simulink model "SWC_FDC_type"  (R2021b)
settings: Solver=FixedStepDiscrete  StartTime=0.0  StopTime=10.0  FixedStep=0.001  RelTol=1e-3
values from neighbouring files (symbols this model uses):
  DID_VCUKey = uint16(0x0202)    [vcu_local_hdr.m]
  DID_XWD = uint16(513)    [vcu_local_hdr.m]
  DIDLen_DKCKey = uint16(8)    [vcu_local_hdr.m]
  DIDLen_DynoMode = uint16(1)    [vcu_local_hdr.m]
  DIDLen_LFLowPresThre = uint16(1)    [vcu_local_hdr.m]
  DIDLen_LFSensorID = uint16(4)    [vcu_local_hdr.m]
  DIDLen_LRLowPresThre = uint16(1)    [vcu_local_hdr.m]
  DIDLen_LRSensorID = uint16(4)    [vcu_local_hdr.m]
  DIDLen_RFLowPresThre = uint16(1)    [vcu_local_hdr.m]
  DIDLen_RFSensorID = uint16(4)    [vcu_local_hdr.m]
  DIDLen_RRLowPresThre = uint16(1)    [vcu_local_hdr.m]
  DIDLen_RRSensorID = uint16(4)    [vcu_local_hdr.m]
  DIDLen_SensorMode = uint16(1)    [vcu_local_hdr.m]
  DIDLen_TPMSLearnSta = uint16(1)    [vcu_local_hdr.m]
  DIDLen_WhlPres = uint16(4)    [vcu_local_hdr.m]
  DIDLen_WhlSensorBattSta = uint16(1)    [vcu_local_hdr.m]
  DIDLen_WhlTmp = uint16(4)    [vcu_local_hdr.m]
  DIDLen_XWDMode = uint16(1)    [vcu_local_hdr.m]
  DIDNum_DKCKey = uint16(0x0202)    [vcu_local_hdr.m]
  DIDNum_DynoMode = uint16(0x0203)    [vcu_local_hdr.m]
  DIDNum_LFLowPresThre = uint16(0x0B08)    [vcu_local_hdr.m]
  DIDNum_LFSensorID = uint16(0x0B01)    [vcu_local_hdr.m]
  DIDNum_LRLowPresThre = uint16(0x0B0A)    [vcu_local_hdr.m]
  DIDNum_LRSensorID = uint16(0x0B03)    [vcu_local_hdr.m]
  DIDNum_RFLowPresThre = uint16(0x0B09)    [vcu_local_hdr.m]
  DIDNum_RFSensorID = uint16(0x0B02)    [vcu_local_hdr.m]
  DIDNum_RRLowPresThre = uint16(0x0B0B)    [vcu_local_hdr.m]
  DIDNum_RRSensorID = uint16(0x0B04)    [vcu_local_hdr.m]
  DIDNum_SensorMode = uint16(0x0B0C)    [vcu_local_hdr.m]
  DIDNum_TPMSLearnSta = uint16(0x0B0D)    [vcu_local_hdr.m]
  DIDNum_WhlPres = uint16(0x0B05)    [vcu_local_hdr.m]
  DIDNum_WhlSensorBattSta = uint16(0x0B07)    [vcu_local_hdr.m]
  DIDNum_WhlTmp = uint16(0x0B06)    [vcu_local_hdr.m]
  DIDNum_XWDMode = uint16(0x0201)    [vcu_local_hdr.m]
  DIDVCUKeyLength = uint16(8)    [vcu_local_hdr.m]
  ENUM_DRIVETRAIN_AWD = uint8(  2  )    [vcu_local_hdr.m]
  ENUM_DRIVETRAIN_FWD = uint8(  1  )    [vcu_local_hdr.m]
  ENUM_DRIVETRAIN_RWD = uint8(  0  )    [vcu_local_hdr.m]
  ENUM_TPMSLearnStatus_LEARNED = uint8(  1  )    [vcu_local_hdr.m]
  ENUM_TPMSLearnStatus_LEARNFAIL = uint8(  2  )    [vcu_local_hdr.m]
  ENUM_TPMSLearnStatus_NOTLEARN = uint8(  0  )    [vcu_local_hdr.m]
  ENUM_TPMSSTA_FAT = uint8(  8  )    [vcu_local_hdr.m]
  ENUM_TPMSSTA_LOWBATTERY = uint8(  2  )    [vcu_local_hdr.m]
  FALSE = boolean( 0 )    [vcu_local_hdr.m]
  ONE_INT = uint8(1)    [vcu_local_hdr.m]
  P_boolean = 0.0    [APPTypes.sldd]
  TRUE = boolean( 1 )    [vcu_local_hdr.m]
  ZERO_FLOAT = single(0)    [vcu_local_hdr.m]
  ZERO_INT = uint8(0)    [vcu_local_hdr.m]
undefined symbols (not defined in the file or in its folder): f32_ApsOutVehSpdSig, KHAL_DKCDecryptEnable_flg_ovrdflg, KHAL_DKCDecryptEnable_flg_ovrdval, KHAL_RandomNumberY1_enum, KHAL_RandomNumberY2_enum, KHAL_RandomNumberY_ovrdflg, KHAL_TPMSRESBUTT_flg_ovrdflg, KHAL_TPMSRESBUTT_flg_ovrdval, R_DIDWriteCDD_CSOP_DIDSet_DKCKey, R_DIDWriteCDD_CSOP_DIDSet_DynoMode, R_DIDWriteCDD_CSOP_DIDSet_LFLowPresThre, R_DIDWriteCDD_CSOP_DIDSet_LFSensorID, R_DIDWriteCDD_CSOP_DIDSet_LRLowPresThre, R_DIDWriteCDD_CSOP_DIDSet_LRSensorID, R_DIDWriteCDD_CSOP_DIDSet_RFLowPresThre, R_DIDWriteCDD_CSOP_DIDSet_RFSensorID, R_DIDWriteCDD_CSOP_DIDSet_RRLowPresThre, R_DIDWriteCDD_CSOP_DIDSet_RRSensorID, R_DIDWriteCDD_CSOP_DIDSet_SensorMode, R_DIDWriteCDD_CSOP_DIDSet_TPMSLearnSta, R_DIDWriteCDD_CSOP_DIDSet_WhlPres, R_DIDWriteCDD_CSOP_DIDSet_WhlSensorBattSta, R_DIDWriteCDD_CSOP_DIDSet_WhlTmp, R_DIDWriteCDD_CSOP_DIDSet_XWDMode, R_E2E_CAN3_VCU1_CSOP_Write_CAN3_VCU1, R_E2E_CAN4_VCU1_CSOP_Write_CAN4_VCU1, R_FDCCDD_Inner_CSOP_FDC_AppCallSleep, R_HALIN_IMU_CSOP_IMUSetSta, R_HALINCDD_CSOP_PAS_Handler, R_HALINCDD_CSOP_UDS_Main, R_HALOUT_APS_CSOP_ApsOutput, R_HALOUTCDD_CSOP_AppNmStateReq, R_HALOUTCDD_CSOP_IVIReset, R_HALOUTCDD_CSOP_SetAcoreRebootCmdACK, R_HALOUTCDD_CSOP_SetSysPwrStat, R_HALOUTCDD_CSOP_SleepRequest, R_NVMReadCDD_Inner_NVM_ReadOperation, R_NVMWriteCDD_Inner_NVM_WriteOperation, R_UDSCDD_CSOP_DdmRestartOperationCycle, R_WDGCDD_CSOP_Call_Watchdog, R_WDGCDD_CSOP_Call_WDG_AppEnd, R_WDGCDD_CSOP_Call_WDG_AppStart, u16_DIDLen_DKCKey, u16_DIDLen_DynoMode, u16_DIDLen_LFLowPresThre, u16_DIDLen_LFSensorID, u16_DIDLen_LRLowPresThre, u16_DIDLen_LRSensorID, u16_DIDLen_RFLowPresThre, u16_DIDLen_RFSensorID, u16_DIDLen_RRLowPresThre, u16_DIDLen_RRSensorID, u16_DIDLen_SensorMode, u16_DIDLen_TPMSLearnSta, u16_DIDLen_WhlPres, u16_DIDLen_WhlSensorBattSta, u16_DIDLen_WhlTmp, u16_DIDLen_XWDMode, u16_DIDNum_DKCKey, u16_DIDNum_DynoMode ... (+42)
libraries: simulink x215, FVT_lib x137, hcu_lib x12, hdlsllib x9, app x1, halin x1, halout x1, inp x1, outp x1
(part 2 of 11)

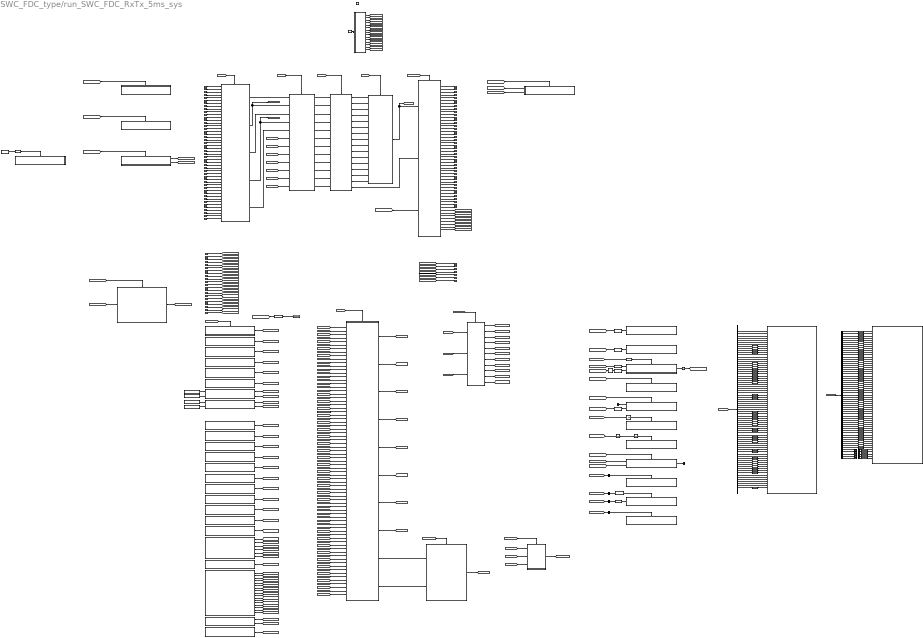
== system SWC_FDC_type/run_SWC_FDC_RxTx_5ms_sys ==
  R_CAN1_ABM1_CAN1_SG_ABM1_read : Inport
  R_CAN1_EPAS1_CAN1_SG_EPAS1_read : Inport  Port=2
  R_CAN1_EPAS2_CAN1_SG_EPAS2_read : Inport  Port=3
  R_CAN1_EPB1_CAN1_SG_EPB1_read : Inport  Port=4
  R_CAN1_ESC1_CAN1_SG_ESC1_read : Inport  Port=5
  R_CAN1_ESC2_CAN1_SG_ESC2_read : Inport  Port=6
  R_CAN1_ESC3_CAN1_SG_ESC3_read : Inport  Port=7
  R_CAN1_ESC4_CAN1_SG_ESC4_read : Inport  Port=8
  R_CAN1_ESC5_CAN1_SG_ESC5_read : Inport  Port=9
  R_CAN1_ESC6_CAN1_SG_ESC6_read : Inport  Port=10
  R_CAN1_ESC7_CAN1_SG_ESC7_read : Inport  Port=11
  R_CAN1_FCM2_CAN1_SG_FCM2_read : Inport  Port=12
  R_CAN1_FCM3_CAN1_SG_FCM3_read : Inport  Port=13
  R_CAN1_FCM4_CAN1_SG_FCM4_read : Inport  Port=14
  R_CAN1_SRR1_CAN1_SG_SRR1_read : Inport  Port=15
  R_CAN2_IVI1_CAN2_SG_IVI1_read : Inport  Port=16
  R_CAN2_IVI2_CAN2_SG_IVI2_read : Inport  Port=17
  R_CAN2_IVI6_CAN2_SG_IVI6_read : Inport  Port=18
  R_CAN2_METER1_CAN2_SG_METER1_read : Inport  Port=19
  R_CAN3_BMS1_CAN3_SG_BMS1_read : Inport  Port=20
  R_CAN3_BMS2_CAN3_SG_BMS2_read : Inport  Port=21
  R_CAN3_BMS3_CAN3_SG_BMS3_read : Inport  Port=22
  R_CAN3_BMS4_CAN3_SG_BMS4_read : Inport  Port=23
  R_CAN3_BMS6_CAN3_SG_BMS6_read : Inport  Port=24
  R_CAN3_BMS7_CAN3_SG_BMS7_read : Inport  Port=25
  R_CAN3_CCU1_CAN3_SG_CCU1_read : Inport  Port=26
  R_CAN3_CCU2_CAN3_SG_CCU2_read : Inport  Port=27
  R_CAN3_CCU4_CAN3_SG_CCU4_read : Inport  Port=28
  R_CAN3_MCU_F1_CAN3_SG_MCU_F1_read : Inport  Port=29
  R_CAN3_MCU_F2_CAN3_SG_MCU_F2_read : Inport  Port=30
  R_CAN3_MCU_R1_CAN3_SG_MCU_R1_read : Inport  Port=31
  R_CAN3_MCU_R2_CAN3_SG_MCU_R2_read : Inport  Port=32
  R_CAN3_Shifter1_CAN3_SG_Shifter1_read : Inport  Port=33
  R_CAN4_DKC1_CAN4_SG_DKC1_read : Inport  Port=34
  R_CAN4_DKC2_CAN4_SG_DKC2_read : Inport  Port=35
  R_CAN4_GW_ZDR_PTG1_CAN4_SG_GW_ZDR_PTG1_read : Inport  Port=36
  R_CAN4_GW_ZoneDR1_CAN4_SG_GW_ZoneDR1_read : Inport  Port=37
  R_CAN4_GW_ZoneDR2_CAN4_SG_GW_ZoneDR2_read : Inport  Port=38
  R_CAN4_GW_ZoneDR3_CAN4_SG_GW_ZoneDR3_read : Inport  Port=39
  R_CAN4_GW_ZoneDR4_CAN4_SG_GW_ZoneDR4_read : Inport  Port=40
  R_CAN4_GW_ZoneDR6_CAN4_SG_GW_ZoneDR6_read : Inport  Port=41
  R_CAN4_GW_ZoneFR1_CAN4_SG_GW_ZoneFR1_read : Inport  Port=42
  R_CAN4_GW_ZoneFR2_CAN4_SG_GW_ZoneFR2_read : Inport  Port=43
  R_CAN4_Zone_Dr_SCP_CAN4_SG_Zone_Dr_SCP_read : Inport  Port=44
  R_CAN4_Zone_Dr_THCM_CAN4_SG_Zone_Dr_THCM_read : Inport  Port=45
  R_CAN4_Zone_Dr_VCU_CAN4_SG_Zone_Dr_VCU_read : Inport  Port=46
  R_CAN4_Zone_Fr_THCM_CAN4_SG_Zone_Fr_THCM_read : Inport  Port=47
  R_CAN5_TBOX1_CAN5_SG_TBOX1_read : Inport  Port=48
  IRV_u16Array4_ApsInDist_read : Inport  Port=49
  IRV_u8Array12_ApsInUssSta_read : Inport  Port=50
  IRV_u8Array256_NvmReadArray_read : Inport  Port=51
  IRV_u8Array8_ApsInLevel_read : Inport  Port=52
  IRV_u8Array8_PasInDist_read : Inport  Port=53
  IRV_u8Array9_TPMSData_read : Inport  Port=54
  IRV_u8_ApsInPASChime_read : Inport  Port=55
  IRV_u8_ApsInSensorLayout_read : Inport  Port=56
  IRV_u8_ApsInSysFailSta_read : Inport  Port=57
  IRV_u8_ApsInSysMode_read : Inport  Port=58
  IRV_u8_CTDSW_read : Inport  Port=59
  IRV_u8_CrashSignal_read : Inport  Port=60
  IRV_u8_DrDoorSW_read : Inport  Port=61
  IRV_u8_HazardSW_read : Inport  Port=62
  IRV_u8_HoodSW_read : Inport  Port=63
  IRV_u8_PsDoorSW_read : Inport  Port=64
  IRV_u8_RLDoorSW_read : Inport  Port=65
  IRV_u8_RRDoorSW_read : Inport  Port=66
  IRV_u8_SeatSW_read : Inport  Port=67
  IRV_u8_TPMSDataInSta_read : Inport  Port=68
  IRV_u8_TailgateSW_read : Inport  Port=69
  IRV_u8_TrunkHanSW_read : Inport  Port=70
  function : TriggerPort  TriggerType=function-call  VariantControl=(inherit)  SampleTimeType=periodic  SampleTime=-1
  APP : app/APP  SystemSampleTime=-1  VariantActivationTime=update diagram  Latency=0  AutoFrameSizeCalculation=off
  Bus Selector : BusSelector  OutputSignals=VOUTP_EnterNewOperCyc_flg
  Bus Selector1 : BusSelector  OutputSignals=VOUTP_AcoreRebootCmdACK_flg
  Bus Selector2 : BusSelector  OutputSignals=VOUTP_IMUEnaCmd_flg
  Bus Selector3 : BusSelector  OutputSignals=VOUTP_PowerSta_enum,VOUTP_BrkPedalPos_pct,VOUTP_ActAPSPosn_pct,VOUTP_LFRawWhlSpeed_kph,VOUTP_RFRawWhlSpeed_kph,VOUTP_LRRawWhlSpeed_kph,VOUTP_RRRawWhlSpeed_kph,VOUTP_LFRawWhlSpeedV_flg,VOUTP_RFRawWhlSpeedV_flg,VOUTP_LRRawWhlSpeedV_flg,VOUTP_RRRawWhlSpeedV_flg,VOUTP_LFWhlRotDir_enum,VOUTP_RFWhlRotDir_enum,VOUTP_LRWhlRotDir_enum,VOUTP_RRWhlRotDir_enum,VOUTP_LFPulseCountV_flg,VOUTP_RFPulseCountV_flg,VOUTP_LRPulseCountV_flg,VOUTP_RRPulseCountV_flg,VOUTP_LFPulseCount_enum,VOUTP_RFPulseCount_enum,VOUTP_LRPulseCount_enum,VOUTP_RRPulseCount_enum,VOUTP_APSActive_flg,VOUTP_APSCtrlAvail_flg,VOUTP_ShifterHandleCmd_enum,VOUTP_DriIntend_enum,VOUTP_EPSAOIControl_enum,VOUTP_SASAngle_Deg,VOUTP_SASSpeed_degps,VOUTP_SASSpeedValid_flg,VOUTP_SASCAL_flg,VOUTP_SASV_flg,VOUTP_GRADE_Deg,VOUTP_YawRate_degps,VOUTP_LatAccel_Gps,VOUTP_LongAccel_Gps,VOUTP_MCPressure_bar,VOUTP_YawRateV_flg,VOUTP_LatAccelV_flg,VOUTP_LongAccelV_flg,VOUTP_MCPressureV_bar,VOUTP_BrkSwSta_flg,VOUTP_BrkSwV_flg,VOUTP_ESCStandstill_flg,VOUTP_ESCAPSSta_enum,VOUTP_EPBExtReleaseAvail_flg,VOUTP_EPBExtApplyAvail_flg,VOUTP_EPBErrSta_enum,VOUTP_EPBSta_enum,VOUTP_AllDoorSW_flg,VOUTP_HoodSW_flg,VOUTP_TailgateSW_flg,VOUTP_AVMparkingcancel_enum,VOUTP_AVMparkingexcute_enum,VOUTP_AVMParkingmode_enum,VOUTP_AVMErrSTA_flg,VOUTP_IVIStatus_flg,VOUTP_CAASSw_enum,VOUTP_IVIScreen_enum,VOUTP_CAASCtrlAvail_flg,VOUTP_ABSActive_flg,VOUTP_TCSActive_flg,VOUTP_DriverSeatBeltCmd_flg,VOUTP_DrDoorSW_flg,VOUTP_PsDoorSW_flg,VOUTP_RLDoorSW_flg,VOUTP_RRDoorSW_flg,VOUTP_RFPressIndi_enum,VOUTP_LFPressIndi_enum,VOUTP_RRPressIndi_enum,VOUTP_LRPressIndi_enum,VOUTP_sigAmbAirT_C,VOUTP_VehActSpd_kph,VOUTP_CAASActive_flg
  Bus Selector4 : BusSelector  OutputSignals=VOUTP_BrkPedalPosTimeOut_flg,VOUTP_LFRawWhlSpeedTimeOut_flg,VOUTP_RFRawWhlSpeedTimeOut_flg,VOUTP_LRRawWhlSpeedTimeOut_flg,VOUTP_RRRawWhlSpeedTimeOut_flg,VOUTP_LFRawWhlSpeedVTimeOut_flg,VOUTP_RFRawWhlSpeedVTimeOut_flg,VOUTP_LRRawWhlSpeedVTimeOut_flg,VOUTP_RRRawWhlSpeedVTimeOut_flg,VOUTP_LFWhlRotDirTimeOut_flg,VOUTP_RFWhlRotDirTimeOut_flg,VOUTP_LRWhlRotDirTimeOut_flg,VOUTP_RRWhlRotDirTimeOut_flg,VOUTP_LFPulseCountVTimeOut_flg,VOUTP_RFPulseCountVTimeOut_flg,VOUTP_LRPulseCountVTimeOut_flg,VOUTP_RRPulseCountVTimeOut_flg,VOUTP_LFPulseCountTimeOut_flg,VOUTP_RFPulseCountTimeOut_flg,VOUTP_LRPulseCountTimeOut_flg,VOUTP_RRPulseCountTimeOut_flg,VOUTP_ShifterHandleCmdTimeOut_flg,VOUTP_DriIntendTimeOut_flg,VOUTP_EPSAOIControlTimeOut_flg,VOUTP_SASAngleTimeOut_flg,VOUTP_SASSpeedTimeOut_flg,VOUTP_SASSpeedValidTimeOut_flg,VOUTP_SASCALTimeOut_flg,VOUTP_SASVTimeOut_flg,VOUTP_GRADETimeOut_flg,VOUTP_YawRateTimeOut_flg,VOUTP_LatAccelTimeOut_flg,VOUTP_LongAccelTimeOut_flg,VOUTP_MCPressureTimeOut_flg,VOUTP_YawRateVTimeOut_flg,VOUTP_LatAccelVTimeOut_flg,VOUTP_LongAccelVTimeOut_flg,VOUTP_MCPressureVTimeOut_flg,VOUTP_BrkSwStaTimeOut_flg,VOUTP_BrkSwVTimeOut_flg,VOUTP_ESCStandstillTimeOut_flg,VOUTP_ESCAPSStaTimeOut_flg,VOUTP_EPBExtReleaseAvailTimeOut_flg,VOUTP_EPBExtApplyAvailTimeOut_flg,VOUTP_EPBErrStaTimeOut_flg,VOUTP_EPBStaTimeOut_flg,VOUTP_AVMparkingcancelTimeOut_flg,VOUTP_AVMparkingexcuteTimeOut_flg,VOUTP_AVMParkingmodeTimeOut_flg,VOUTP_AVMErrSTATimeOut_flg,VOUTP_IVIStatusTimeOut_flg,VOUTP_CAASSwTimeOut_flg,VOUTP_IVIScreenTimeOut_flg,VOUTP_ABSActiveTimeOut_flg,VOUTP_TCSActiveTimeOut_flg,VOUTP_DriverSeatBeltCmdTimeOut_flg,VOUTP_RFPressIndi_enum,VOUTP_LFPressIndi_enum,VOUTP_RRPressIndi_enum,VOUTP_LRPressIndi_enum,VOUTP_sigAmbAirT_C
  Bus Selector5 : BusSelector  OutputSignals=VOUTP_IMUEnaCmd_flg
  Constant : Constant  Value=DIDVCUKeyLength
  Constant1 : Constant  Value=DID_VCUKey
  Constant2 : Constant  Value=uint16(ONE_INT)
  Constant3 : Constant  Value=DID_XWD
  Constant4 : Constant  Value=TRUE
  Constant5 : Constant  Value=FALSE
  Constant6 : Constant  Value=ONE_INT
  DID_CDDSubsystem : Subsystem
  Data Type Conversion{,1..3,5..13,17..19,21..96,98..106,123} (102 alike) : DataTypeConversion  OutDataTypeStr=uint8
  Data Type Conversion{14..16,20} (4 alike) : DataTypeConversion  OutDataTypeStr=int16
  Data Type Conversion4 : DataTypeConversion  OutDataTypeStr=uint32
  Display : Display
  Ground{,1..5} (6 alike) : Ground
  HALOUT_AFTER : Subsystem
  HAL_IN : halin/HAL_IN  SystemSampleTime=-1  VariantActivationTime=update diagram  Latency=0  AutoFrameSizeCalculation=off
  HAL_OUT : halout/HAL_OUT  SystemSampleTime=-1  VariantActivationTime=update diagram  Latency=0  AutoFrameSizeCalculation=off
  Halin_CDD : Subsystem
      settings: RTWSystemCode=Nonreusable function  RTWFcnNameOpts=Use subsystem name  RTWFileNameOpts=Use subsystem name
  INP : inp/INP  SystemSampleTime=-1  VariantActivationTime=update diagram  Latency=0  AutoFrameSizeCalculation=off
  Latch : hcu_lib/Basic_Blocks/Latch
  NOT : Logic  Operator=NOT  Inputs=1  AllPortsSameDT=off  OutDataTypeStr=boolean
  OUTP : outp/OUTP  SystemSampleTime=-1  VariantActivationTime=update diagram  Latency=0  AutoFrameSizeCalculation=off
  OUTP_AFTER : Subsystem
      settings: RTWSystemCode=Nonreusable function  RTWFcnNameOpts=Use subsystem name  RTWFileNameOpts=Use subsystem name
  R_FDCCDD_Inner_CSOP_FDC_AppCallSleep : Subsystem
  R_HALINCDD_CSOP_CAN1BusOff : FunctionCaller  FunctionPrototype=u8_CAN1BusOff = R_HALINCDD_CSOP_CAN1BusOff()  OutputArgumentSpecifications=uint8(1)
  R_HALINCDD_CSOP_CAN2BusOff : FunctionCaller  FunctionPrototype=u8_CAN2BusOff = R_HALINCDD_CSOP_CAN2BusOff()  OutputArgumentSpecifications=uint8(1)
  R_HALINCDD_CSOP_CAN3BusOff : FunctionCaller  FunctionPrototype=u8_CAN3BusOff = R_HALINCDD_CSOP_CAN3BusOff()  OutputArgumentSpecifications=uint8(1)
  R_HALINCDD_CSOP_CAN4BusOff : FunctionCaller  FunctionPrototype=u8_CAN4BusOff = R_HALINCDD_CSOP_CAN4BusOff()  OutputArgumentSpecifications=uint8(1)
  R_HALINCDD_CSOP_CAN5BusOff : FunctionCaller  FunctionPrototype=u8_CAN5BusOff = R_HALINCDD_CSOP_CAN5BusOff()  OutputArgumentSpecifications=uint8(1)
  R_HALINCDD_CSOP_DIDgetDKCdata : FunctionCaller  FunctionPrototype=[u8_DidStaDKC,u8Array8_DidDataDKC] = R_HALINCDD_CSOP_DIDgetDKCdata(u16_lengthDIDDKC,u16_DIDDKC)  InputArgumentSpecifications=uint16(1), uint16(1)  OutputArgumentSpecifications=uint8(1), uint8([1;1;1;1;1;1;1;1])
  R_HALINCDD_CSOP_DIDgetXWDdata : FunctionCaller  FunctionPrototype=[u8_DidStaXWD,u8_DidDataXWD] = R_HALINCDD_CSOP_DIDgetXWDdata(u16_lengthDIDXWD,u16_DIDXWD)  InputArgumentSpecifications=uint16(1), uint16(1)  OutputArgumentSpecifications=uint8(1), uint8(1)
  R_HALINCDD_CSOP_GetAcoreReadyToSleep : FunctionCaller  FunctionPrototype=s8_AcoreReadyToSleep = R_HALINCDD_CSOP_GetAcoreReadyToSleep()  OutputArgumentSpecifications=int8(1)
  R_HALINCDD_CSOP_GetAcoreRebootCmd : FunctionCaller  FunctionPrototype=u8_AcoreRebootCmd = R_HALINCDD_CSOP_GetAcoreRebootCmd()  OutputArgumentSpecifications=uint8(1)
  R_HALINCDD_CSOP_GetAuxBattVoltage : FunctionCaller  FunctionPrototype=u16_AuxBattVol100mV = R_HALINCDD_CSOP_GetAuxBattVoltage()  OutputArgumentSpecifications=uint16(1)
  R_HALINCDD_CSOP_GetBootReason : FunctionCaller  FunctionPrototype=u8_BootReason = R_HALINCDD_CSOP_GetBootReason()  OutputArgumentSpecifications=uint8(1)
  R_HALINCDD_CSOP_GetEvccAplusPwrUpReq : FunctionCaller  FunctionPrototype=u8_EvccAplusPwrUpReq = R_HALINCDD_CSOP_GetEvccAplusPwrUpReq()  OutputArgumentSpecifications=uint8(1)
  R_HALINCDD_CSOP_GetNmState : FunctionCaller  FunctionPrototype=u8_CurrentNMState = R_HALINCDD_CSOP_GetNmState()  OutputArgumentSpecifications=uint8(1)
  R_HALINCDD_CSOP_GetNvmProtectState : FunctionCaller  FunctionPrototype=u8_NvmProtectSta = R_HALINCDD_CSOP_GetNvmProtectState()  OutputArgumentSpecifications=uint8(1)
  R_HALINCDD_CSOP_GetSWID : FunctionCaller  FunctionPrototype=u8Array33_SWID = R_HALINCDD_CSOP_GetSWID()  OutputArgumentSpecifications=uint8([1;1;1;1;1;1;1;1;1;1;1;1;1;1;1;1;1;1;1;1;1;1;1;1;1;1;1;1;1;1;1;1;1])
  R_HALINCDD_CSOP_GetVinpAllowMoveThdOta : FunctionCaller  FunctionPrototype=u8_AllowMovThdOTA = R_HALINCDD_CSOP_GetVinpAllowMoveThdOta()  OutputArgumentSpecifications=uint8(1)
  R_HALINCDD_CSOP_GetVinpPwrReqOta : FunctionCaller  FunctionPrototype=u8_PwrReqOTA = R_HALINCDD_CSOP_GetVinpPwrReqOta()  OutputArgumentSpecifications=uint8(1)
  R_HALINCDD_CSOP_GetWISR : FunctionCaller  FunctionPrototype=u32_WISR = R_HALINCDD_CSOP_GetWISR()  OutputArgumentSpecifications=uint32(1)
  R_HALINCDD_CSOP_HALINCDD_DIRECT : FunctionCaller  FunctionPrototype=[u8_BrakeSW,u8_BrakeLamp,u16_Pedal1Vol,u16_Pedal2Vol,u16_Pedal1Ref5V,u16_Pedal2Ref5V] = R_HALINCDD_CSOP_HALINCDD_DIRECT()  OutputArgumentSpecifications=uint8(1), uint8(1), uint16(1), uint16(1), uint16(1), uint16(1)
  R_HALINCDD_u8Array4_HWID : FunctionCaller  FunctionPrototype=u8Array4_HWID = R_HALINCDD_u8Array4_HWID()  OutputArgumentSpecifications=uint8([1;1;1;1])
  R_HALIN_APS_CSOP_ApsGetData : FunctionCaller  FunctionPrototype=[u8_GetAPS_Progress_PCT,u8_GetAPS_RQ_Display,u8_GetAPS_SW_Ver,u8_GetAPS_HW_Ver,u8_GetAPS_ExitCondition,f32_GetAPS_Angle_Target,u8_GetAPS_Sta_System,u8_GetAPS_V_Rq_EPAS_Ctrl,u8_GetAPS_Rq_EPAS_Ctrl,u8_GetAPS_Req,f32_GetAPS_DecReq,u8_GetAPS_DecReq_A,f32_GetAPS_SpeedCmd,u8_GetAPS_ShftPosnReq,u8_GetAPS_VMC_Req_A,u8_GetCAAS_Sta,u8_GetCAAS_VMC_Req_A] = R_HALIN_APS_CSOP_ApsGetData()  OutputArgumentSpecifications=uint8(1), uint8(1), uint8(1), uint8(1), uint8(1), single(1), uint8(1), uint8(1), uint8(1), uint8(1), single(1), uint8(1), single(1), uint8(1), uint8(1), uint8(1), uint8(1)
  R_HALIN_IMU_CSOP_IMUGetOffsetVal : Subsystem
  R_HALIN_IMU_CSOP_IMUGetSixAxisVal : FunctionCaller  FunctionPrototype=[s16_IMUSixAxisVal,u8_IMUSixAxisValSta] = R_HALIN_IMU_CSOP_IMUGetSixAxisVal()  OutputArgumentSpecifications=int16([1;1;1;1;1;1]), uint8(1)
  R_HALIN_IMU_CSOP_IMUSetSta : Subsystem
  R_HALOUTCDD_CSOP_AppNmStateReq : Subsystem
  R_HALOUTCDD_CSOP_IVIReset : FunctionCaller  FunctionPrototype=R_HALOUTCDD_CSOP_IVIReset(u8_RstValue)  InputArgumentSpecifications=uint8(1)
  R_HALOUTCDD_CSOP_SetAcoreRebootCmdACK : Subsystem
  R_HALOUTCDD_CSOP_SetSysPwrStat : FunctionCaller  FunctionPrototype=R_HALOUTCDD_CSOP_SetSysPwrStat(u8_SysPwrStat)  InputArgumentSpecifications=uint8(1)
  R_HALOUTCDD_CSOP_SleepRequest : Subsystem
  R_HALOUT_APS_CSOP_ApsSetData : FunctionCaller  FunctionPrototype=R_HALOUT_APS_CSOP_ApsSetData(u8_SetPwrSta,f32_SetBrkPedalPos,f32_SetActAPSPosn,f32_SetLF_RawWhlSpeed,f32_SetRF_RawWhlSpeed,f32_SetLR_RawWhlSpeed,f32_SetRR_RawWhlSpeed,u8_SetLF_RawWhlSpeed_V,u8_SetRF_RawWhlSpeed_V,u8_SetLR_RawWhlSpeed_V,u8_SetRR_RawWhlSpeed_V,u8_SetLF_WhlRotDir,u8_SetRF_WhlRotDir,u8_SetLR_WhlRotDir,u8_SetRR_WhlRotDir,u8_SetLF_PulseCount_V,u8_SetRF_PulseCount_V,u8_SetLR_PulseCount_V,u8_SetRR_PulseCount_V,s16_SetLF_PulseCount,s16_SetRF_PulseCount,s16_SetLR_PulseCount,s16_SetRR_PulseCount,u8_SetAPS_Active,u8_SetAPS_CtrlAvail,u8_SetShifter_Handle_Cmd,u8_SetDriIntend,u8_SetEPS_AOI_Control,f32_SetSAS_Angle,f32_SetSAS_Speed,u8_SetSAS_Speed_Valid,u8_SetSAS_CAL,u8_SetSAS_OK,f32_SetGRADE,f32_SetYawRate,f32_SetLatAccel,f32_SetLongAccel,f32_SetMCPressure,u8_SetYawRate_V,u8_SetLatAccel_V,u8_SetLongAccel_V,u8_SetMCPressure_V,u8_SetBrkSw_Sta,u8_SetBrkSw_V,u8_SetESC_Standstill,u8_SetESC_APS_Sta,u8_SetEPBExtReleaseAvail,u8_SetEPBExtApplyAvail,u8_SetEPBErrSta,u8_SetEPBSta,u8_SetAllDoorSW,u8_SetHoodSW,u8_SetTailgate_SW,u8_SetAVM_parking_cancel,u8_SetAVM_parking_excute,u8_SetAVM_Parking_mode,u8_SetAVM_Err_STA,u8_SetIVI_Status,u8_SetCAAS_Sw,u8_SetIVI_Screen,u8_SetCAAS_CtrlAvail,u8_SetABS_Active,u8_SetTCS_Active,u8_SetDriverSeatBeltCmd,u8_SetDrDoorSW,u8_SetPsDoorSW,u8_SetRLDoorSW,u8_SetRRDoorSW,u8_SetRFPressIndi,u8_SetLFPressIndi,u8_SetRRPressIndi,u8_SetLRPressIndi,f32_SetsigAmbAirT,f32_SetVehActSpd,u8_SetCAAS_Active)  InputArgumentSpecifications=uint8(1), single(1), single(1), single(1), single(1), single(1), single(1), uint8(1), uint8(1), uint8(1), uint8(1), uint8(1), uint8(1), uint8(1), uint8(1), uint8(1), uint8(1), uint8(1), uint8(1), int16(1), int16(1), int16(1), int16(1), uint8(1), uint8(1), uint8(1), uint8(1), uint8(1), single(1), single(1), uint8(1), uint8(1), uint8(1), single(1), single(1), single(1), single(1), single(1), uint8(1), uint8(1), uint8(1), uint8(1), uint8(1), uint8(1), uint8(1), uint8(1), uint8(1), uint8(1), uint8(1), uint8(1), uint8(1), uint8(1), uint8(1), uint8(1), uint8(1), uint8(1), uint8(1), uint8(1), uint8(1), uint8(1), uint8(1), uint8(1), uint8(1), uint8(1), uint8(1), uint8(1), uint8(1), uint8(1), uint8(1), uint8(1), uint8(1), uint8(1), single(1), single(1), uint8(1)
  R_HALOUT_APS_CSOP_ApsSetTimeout : FunctionCaller  FunctionPrototype=R_HALOUT_APS_CSOP_ApsSetTimeout(u8_SetBrkPedalPosTO,u8_SetLF_RawWhlSpeedTO,u8_SetRF_RawWhlSpeedTO,u8_SetLR_RawWhlSpeedTO,u8_SetRR_RawWhlSpeedTO,u8_SetLF_RawWhlSpeed_VTO,u8_SetRF_RawWhlSpeed_VTO,u8_SetLR_RawWhlSpeed_VTO,u8_SetRR_RawWhlSpeed_VTO,u8_SetLF_WhlRotDirTO,u8_SetRF_WhlRotDirTO,u8_SetLR_WhlRotDirTO,u8_SetRR_WhlRotDirTO,u8_SetLF_PulseCount_VTO,u8_SetRF_PulseCount_VTO,u8_SetLR_PulseCount_VTO,u8_SetRR_PulseCount_VTO,u8_SetLF_PulseCountTO,u8_SetRF_PulseCountTO,u8_SetLR_PulseCountTO,u8_SetRR_PulseCountTO,u8_SetShifter_Handle_CmdTO,u8_SetDriIntendTO,u8_SetEPS_AOI_ControlTO,u8_SetSAS_AngleTO,u8_SetSAS_SpeedTO,u8_SetSAS_Speed_ValidTO,u8_SetSAS_CALTO,u8_SetSAS_OKTO,u8_SetGRADETO,u8_SetYawRateTO,u8_SetLatAccelTO,u8_SetLongAccelTO,u8_SetMCPressureTO,u8_SetYawRate_VTO,u8_SetLatAccel_VTO,u8_SetLongAccel_VTO,u8_SetMCPressure_VTO,u8_SetBrkSw_StaTO,u8_SetBrkSw_VTO,u8_SetESC_StandstillTO,u8_SetESC_APS_StaTO,u8_SetEPBExtReleaseAvailTO,u8_SetEPBExtApplyAvailTO,u8_SetEPBErrStaTO,u8_SetEPBStaTO,u8_SetAVM_parking_cancelTO,u8_SetAVM_parking_excuteTO,u8_SetAVM_Parking_modeTO,u8_SetAVM_Err_STATO,u8_SetIVI_StatusTO,u8_SetCAAS_SwTO,u8_SetIVI_ScreenTO,u8_SetABS_ActiveTO,u8_SetTCS_ActiveTO,u8_SetDriverSeatBeltCmdTO,u8_SetRFPressIndiTO,u8_SetLFPressIndiTO,u8_SetRRPressIndiTO,u8_SetLRPressIndiTO,u8_SetsigAmbAirTTO)  InputArgumentSpecifications=uint8(1), uint8(1), uint8(1), uint8(1), uint8(1), uint8(1), uint8(1), uint8(1), uint8(1), uint8(1), uint8(1), uint8(1), uint8(1), uint8(1), uint8(1), uint8(1), uint8(1), uint8(1), uint8(1), uint8(1), uint8(1), uint8(1), uint8(1), uint8(1), uint8(1), uint8(1), uint8(1), uint8(1), uint8(1), uint8(1), uint8(1), uint8(1), uint8(1), uint8(1), uint8(1), uint8(1), uint8(1), uint8(1), uint8(1), uint8(1), uint8(1), uint8(1), uint8(1), uint8(1), uint8(1), uint8(1), uint8(1), uint8(1), uint8(1), uint8(1), uint8(1), uint8(1), uint8(1), uint8(1), uint8(1), uint8(1), uint8(1), uint8(1), uint8(1), uint8(1), uint8(1)
  R_NVMReadCDD_Inner_NVM_ReadOperation : Subsystem
  R_NVMWriteCDD_Inner_NVM_WriteOperation : Subsystem
  R_UDSCDD_CSOP_DdmClearDTCNotification : FunctionCaller  FunctionPrototype=u8_ClearDTCcmd = R_UDSCDD_CSOP_DdmClearDTCNotification()  OutputArgumentSpecifications=uint8(1)
  R_UDSCDD_CSOP_DdmRestartOperationCycle : Subsystem
  R_UDSCDD_CSOP_SetDTCStatus : Subsystem
  R_WDGCDD_CSOP_Call_WDG_AppEnd : Subsystem
  R_WDGCDD_CSOP_Call_WDG_AppStart : Subsystem
  R_WDGCDD_CSOP_Call_Watchdog : Subsystem
  Real_DetectChange : hcu_lib/Basic_Blocks/Real_DetectChange
  Subsystem : Subsystem
  Subsystem1 : Subsystem
  Subsystem2 : Subsystem
  Terminator{,1..5} (6 alike) : Terminator
  Unit Delay{,1..3} (4 alike) : UnitDelay  SampleTime=-1  HasFrameUpgradeWarning=on
  detect_Increase : simulink/Logic and Bit Operations/Detect Increase  vinit=0.0  OutDataTypeStr=boolean
  detect_change : simulink/Logic and Bit Operations/Detect Change  vinit=0  OutDataTypeStr=boolean
  hcu_main_sched : Stateflow chart  TreatAsAtomicUnit=on
  P_CAN1_FD_BCM1_CAN1_SG_FD_BCM1_write : Outport
  P_CAN1_FD_VCU1_CAN1_SG_FD_VCU1_write : Outport  Port=2
  P_CAN1_FD_VCU4_CAN1_SG_FD_VCU4_write : Outport  Port=3
  P_CAN2_FD_BCM1_CAN2_SG_FD_BCM1_write : Outport  Port=4
  P_CAN2_FD_BCM2_CAN2_SG_FD_BCM2_write : Outport  Port=5
  P_CAN2_FD_TPMS1_CAN2_SG_FD_TPMS1_write : Outport  Port=6
  P_CAN2_FD_TPMS2_CAN2_SG_FD_TPMS2_write : Outport  Port=7
  P_CAN2_FD_V2L1_CAN2_SG_FD_V2L1_write : Outport  Port=8
  P_CAN2_FD_VCU0_CAN2_SG_FD_VCU0_write : Outport  Port=9
  P_CAN2_FD_VCU1_CAN2_SG_FD_VCU1_write : Outport  Port=10
  P_CAN2_FD_VCU4_CAN2_SG_FD_VCU4_write : Outport  Port=11
  P_CAN2_FD_VMC1_CAN2_SG_FD_VMC1_write : Outport  Port=12
  P_CAN3_FD_BCM1_CAN3_SG_FD_BCM1_write : Outport  Port=13
  P_CAN3_FD_THCM2_CAN3_SG_FD_THCM2_write : Outport  Port=14
  P_CAN3_FD_V2L1_CAN3_SG_FD_V2L1_write : Outport  Port=15
  P_CAN4_FD_DKC1_CAN4_SG_FD_DKC1_write : Outport  Port=16
  P_CAN4_FD_THCM2_CAN4_SG_FD_THCM2_write : Outport  Port=17
  P_CAN5_FD_BCM1_CAN5_SG_FD_BCM1_write : Outport  Port=18
  P_CAN5_FD_CONN1_CAN5_SG_FD_CONN1_write : Outport  Port=19
  P_CAN5_FD_THCM2_CAN5_SG_FD_THCM2_write : Outport  Port=20
  P_CAN5_FD_VCU0_CAN5_SG_FD_VCU0_write : Outport  Port=21
  P_CAN5_FD_VCU1_CAN5_SG_FD_VCU1_write : Outport  Port=22
  P_CAN5_FD_VCU4_CAN5_SG_FD_VCU4_write : Outport  Port=23
  IRV_ms10_CAN1_SG_FD_APS3_write : Outport  Port=24  OutDataTypeStr=Bus: DT_CAN1_SG_FD_APS3  PortDimensions=1  BusOutputAsStruct=on
  IRV_ms10_CAN1_SG_FD_VCU2_write : Outport  Port=25  OutDataTypeStr=Bus: DT_CAN1_SG_FD_VCU2  PortDimensions=1  BusOutputAsStruct=on
  IRV_ms10_CAN1_SG_FD_VCU3_write : Outport  Port=26  OutDataTypeStr=Bus: DT_CAN1_SG_FD_VCU3  PortDimensions=1  BusOutputAsStruct=on
  IRV_ms10_CAN2_SG_FD_APS3_write : Outport  Port=27  OutDataTypeStr=Bus: DT_CAN2_SG_FD_APS3  PortDimensions=1  BusOutputAsStruct=on
  IRV_ms10_CAN2_SG_FD_VCU2_write : Outport  Port=28  OutDataTypeStr=Bus: DT_CAN2_SG_FD_VCU2  PortDimensions=1  BusOutputAsStruct=on
  IRV_ms10_CAN3_SG_FD_VCU0_write : Outport  Port=29  OutDataTypeStr=Bus: DT_CAN3_SG_FD_VCU0  PortDimensions=1  BusOutputAsStruct=on
  IRV_ms10_CAN3_SG_FD_VCU2_write : Outport  Port=30  OutDataTypeStr=Bus: DT_CAN3_SG_FD_VCU2  PortDimensions=1  BusOutputAsStruct=on
  IRV_ms10_CAN5_SG_FD_VCU3_write : Outport  Port=31  OutDataTypeStr=Bus: DT_CAN5_SG_FD_VCU3  PortDimensions=1  BusOutputAsStruct=on
  IRV_ms100_CAN1_SG_FD_THCM1_write : Outport  Port=32  OutDataTypeStr=Bus: DT_CAN1_SG_FD_THCM1  PortDimensions=1  BusOutputAsStruct=on
  IRV_ms100_CAN2_SG_FD_THCM1_write : Outport  Port=33  OutDataTypeStr=Bus: DT_CAN2_SG_FD_THCM1  PortDimensions=1  BusOutputAsStruct=on
  IRV_ms100_CAN3_SG_FD_THCM1_write : Outport  Port=34  OutDataTypeStr=Bus: DT_CAN3_SG_FD_THCM1  PortDimensions=1  BusOutputAsStruct=on
  IRV_ms100_CAN4_SG_FD_THCM1_write : Outport  Port=35  OutDataTypeStr=Bus: DT_CAN4_SG_FD_THCM1  PortDimensions=1  BusOutputAsStruct=on
  IRV_ms20_CAN1_SG_FD_APS1_write : Outport  Port=36  OutDataTypeStr=Bus: DT_CAN1_SG_FD_APS1  PortDimensions=1  BusOutputAsStruct=on
  IRV_ms20_CAN1_SG_FD_APS2_write : Outport  Port=37  OutDataTypeStr=Bus: DT_CAN1_SG_FD_APS2  PortDimensions=1  BusOutputAsStruct=on
  IRV_ms20_CAN2_SG_FD_APS1_write : Outport  Port=38  OutDataTypeStr=Bus: DT_CAN2_SG_FD_APS1  PortDimensions=1  BusOutputAsStruct=on
  IRV_ms20_CAN2_SG_FD_APS2_write : Outport  Port=39  OutDataTypeStr=Bus: DT_CAN2_SG_FD_APS2  PortDimensions=1  BusOutputAsStruct=on
  IRV_ms500_CAN2_SG_FD_VCU5_write : Outport  Port=40  OutDataTypeStr=Bus: DT_CAN2_SG_FD_VCU5  PortDimensions=1  BusOutputAsStruct=on
  IRV_ms500_CAN5_SG_FD_VCU5_write : Outport  Port=41  OutDataTypeStr=Bus: DT_CAN5_SG_FD_VCU5  PortDimensions=1  BusOutputAsStruct=on
  IRV_ms5000_CAN2_SG_FD_VCU6_write : Outport  Port=42  OutDataTypeStr=Bus: DT_CAN2_SG_FD_VCU6  PortDimensions=1  BusOutputAsStruct=on
  IRV_E2E_CAN3_SG_FD_VCU1_write : Outport  Port=43  OutDataTypeStr=Bus: DT_CAN3_SG_FD_VCU1  PortDimensions=1  BusOutputAsStruct=on
  IRV_E2E_CAN4_SG_FD_VCU1_write : Outport  Port=44  OutDataTypeStr=Bus: DT_CAN4_SG_FD_VCU1  PortDimensions=1  BusOutputAsStruct=on
  IRV_f32_ApsOutVehSpdSig_write : Outport  Port=45  OutDataTypeStr=single  PortDimensions=1
  IRV_u8Array256_NvmWriteArray_write : Outport  Port=46  OutDataTypeStr=uint8  PortDimensions=256
  IRV_u8_ApsOutGearPosnSig_write : Outport  Port=47  OutDataTypeStr=uint8  PortDimensions=1
  IRV_u8_ApsOutSendChrgPlugSta_write : Outport  Port=48  OutDataTypeStr=uint8  PortDimensions=1
  IRV_u8_ApsOutSetFrSensorOnCmd_write : Outport  Port=49  OutDataTypeStr=uint8  PortDimensions=1
  IRV_u8_ApsOutSetFrSensorSwTOCmd_write : Outport  Port=50  OutDataTypeStr=uint8  PortDimensions=1
  IRV_u8_ApsOutSetVehSpdTOCmd_write : Outport  Port=51  OutDataTypeStr=uint8  PortDimensions=1
  wires:
  IRV_u16Array4_ApsInDist_read/1 -> [u16Array4_ApsInDist]
  IRV_u8Array12_ApsInUssSta_read/1 -> [u8Array12_ApsInUssSta]
  IRV_u8Array256_NvmReadArray_read/1 -> [u8Array256_NvmReadArray]
  IRV_u8Array8_ApsInLevel_read/1 -> [u8Array8_ApsInLevel]
  IRV_u8Array8_PasInDist_read/1 -> [u8Array8_PasInDist]
  IRV_u8Array9_TPMSData_read/1 -> [u8Array9_TPMSData]
  IRV_u8_ApsInPASChime_read/1 -> [u8_ApsInPASChime]
  IRV_u8_ApsInSensorLayout_read/1 -> [u8_ApsInSensorLayout]
  IRV_u8_ApsInSysFailSta_read/1 -> [u8_ApsInSysFailSta]
  IRV_u8_ApsInSysMode_read/1 -> [u8_ApsInSysMode]
  IRV_u8_CTDSW_read/1 -> [u8_CTDSW]
  IRV_u8_CrashSignal_read/1 -> [u8_CrashSignal]
  IRV_u8_DrDoorSW_read/1 -> [u8_DrDoorSW]
  IRV_u8_HazardSW_read/1 -> [u8_HazardSW]
  IRV_u8_HoodSW_read/1 -> [u8_HoodSW]
  IRV_u8_PsDoorSW_read/1 -> [u8_PsDoorSW]
  IRV_u8_RLDoorSW_read/1 -> [u8_RLDoorSW]
  IRV_u8_RRDoorSW_read/1 -> [u8_RRDoorSW]
  IRV_u8_SeatSW_read/1 -> [u8_SeatSW]
  IRV_u8_TPMSDataInSta_read/1 -> [u8_TPMSDataInSta]
  IRV_u8_TailgateSW_read/1 -> [u8_TailgateSW]
  IRV_u8_TrunkHanSW_read/1 -> [u8_TrunkHanSW]
  [f32_ApsOutVehSpdSig] -> IRV_f32_ApsOutVehSpdSig_write/1
  [u8Array256_NvmWriteArray] -> IRV_u8Array256_NvmWriteArray_write/1
  [u8_ApsOutGearPosnSig] -> IRV_u8_ApsOutGearPosnSig_write/1
  [u8_ApsOutSendChrgPlugSta] -> IRV_u8_ApsOutSendChrgPlugSta_write/1
  [u8_ApsOutSetFrSensorOnCmd] -> IRV_u8_ApsOutSetFrSensorOnCmd_write/1
  [u8_ApsOutSetFrSensorSwTOCmd] -> IRV_u8_ApsOutSetFrSensorSwTOCmd_write/1
  [u8_ApsOutSetVehSpdTOCmd] -> IRV_u8_ApsOutSetVehSpdTOCmd_write/1
  R_HALINCDD_CSOP_CAN1BusOff/1 -> [u8_CAN1BusOff]
  R_HALINCDD_CSOP_CAN2BusOff/1 -> [u8_CAN2BusOff]
  R_HALINCDD_CSOP_CAN3BusOff/1 -> [u8_CAN3BusOff]
  R_HALINCDD_CSOP_CAN4BusOff/1 -> [u8_CAN4BusOff]
  R_HALINCDD_CSOP_CAN5BusOff/1 -> [u8_CAN5BusOff]
  Constant/1 -> R_HALINCDD_CSOP_DIDgetDKCdata/1
  Constant1/1 -> R_HALINCDD_CSOP_DIDgetDKCdata/2
  R_HALINCDD_CSOP_DIDgetDKCdata/1 -> [u8_DidStaDKC]
  R_HALINCDD_CSOP_DIDgetDKCdata/2 -> [u8Array8_DidDataDKC]
  Constant2/1 -> R_HALINCDD_CSOP_DIDgetXWDdata/1
  Constant3/1 -> R_HALINCDD_CSOP_DIDgetXWDdata/2
  R_HALINCDD_CSOP_DIDgetXWDdata/1 -> [u8_DidStaXWD]
  R_HALINCDD_CSOP_DIDgetXWDdata/2 -> [u8_DidDataXWD]
  R_HALINCDD_CSOP_GetAcoreReadyToSleep/1 -> [s8_AcoreReadyToSleep]
  R_HALINCDD_CSOP_GetAcoreRebootCmd/1 -> [u8_AcoreRebootCmd]
  R_HALINCDD_CSOP_GetAuxBattVoltage/1 -> [u16_AuxBattVol100mV]
  R_HALINCDD_CSOP_GetBootReason/1 -> [u8_BootReason]
  R_HALINCDD_CSOP_GetEvccAplusPwrUpReq/1 -> [u8_EvccAplusPwrUpReq]
  R_HALINCDD_CSOP_GetNmState/1 -> [u8_CurrentNMState]
  R_HALINCDD_CSOP_GetNvmProtectState/1 -> [u8_NvmProtectSta]
  R_HALINCDD_CSOP_GetSWID/1 -> [u8Array33_SWID]
  R_HALINCDD_CSOP_GetVinpAllowMoveThdOta/1 -> [u8_AllowMovThdOTA]
  R_HALINCDD_CSOP_GetVinpPwrReqOta/1 -> [u8_PwrReqOTA]
  R_HALINCDD_CSOP_GetWISR/1 -> [u32_WISR]
  R_HALINCDD_CSOP_HALINCDD_DIRECT/1 -> [u8_BrakeSW]
  R_HALINCDD_CSOP_HALINCDD_DIRECT/2 -> [u8_BrakeLamp]
  R_HALINCDD_CSOP_HALINCDD_DIRECT/3 -> [u16_Pedal1Vol]
  R_HALINCDD_CSOP_HALINCDD_DIRECT/4 -> [u16_Pedal2Vol]
  R_HALINCDD_CSOP_HALINCDD_DIRECT/5 -> [u16_Pedal1Ref5V]
  R_HALINCDD_CSOP_HALINCDD_DIRECT/6 -> [u16_Pedal2Ref5V]
  R_HALINCDD_u8Array4_HWID/1 -> [u8Array4_HWID]
  R_HALIN_APS_CSOP_ApsGetData/1 -> [u8_GetAPS_Progress_PCT]
  R_HALIN_APS_CSOP_ApsGetData/2 -> [u8_GetAPS_RQ_Display]
  R_HALIN_APS_CSOP_ApsGetData/3 -> [u8_GetAPS_SW_Ver]
  R_HALIN_APS_CSOP_ApsGetData/4 -> [u8_GetAPS_HW_Ver]
  R_HALIN_APS_CSOP_ApsGetData/5 -> [u8_GetAPS_ExitCondition]
  R_HALIN_APS_CSOP_ApsGetData/6 -> [f32_GetAPS_Angle_Target]
  R_HALIN_APS_CSOP_ApsGetData/7 -> [u8_GetAPS_Sta_System]
  R_HALIN_APS_CSOP_ApsGetData/8 -> [u8_GetAPS_V_Rq_EPAS_Ctrl]
  R_HALIN_APS_CSOP_ApsGetData/9 -> [u8_GetAPS_Rq_EPAS_Ctrl]
  R_HALIN_APS_CSOP_ApsGetData/10 -> [u8_GetAPS_Req]
  R_HALIN_APS_CSOP_ApsGetData/11 -> [f32_GetAPS_DecReq]
  R_HALIN_APS_CSOP_ApsGetData/12 -> [u8_GetAPS_DecReq_A]
  R_HALIN_APS_CSOP_ApsGetData/13 -> [f32_GetAPS_SpeedCmd]
  R_HALIN_APS_CSOP_ApsGetData/14 -> [u8_GetAPS_ShftPosnReq]
  R_HALIN_APS_CSOP_ApsGetData/15 -> [u8_GetAPS_VMC_Req_A]
  R_HALIN_APS_CSOP_ApsGetData/16 -> [u8_GetCAAS_Sta]
  R_HALIN_APS_CSOP_ApsGetData/17 -> [u8_GetCAAS_VMC_Req_A]
  R_HALIN_IMU_CSOP_IMUGetSixAxisVal/1 -> [s16_IMUSixAxisVal]
  R_HALIN_IMU_CSOP_IMUGetSixAxisVal/2 -> [u8_IMUSixAxisValSta]
  R_UDSCDD_CSOP_DdmClearDTCNotification/1 -> [u8_ClearDTCcmd]
  Data Type Conversion/1 -> R_HALOUTCDD_CSOP_IVIReset/1
  [VOUTP_IVIRST_flg] -> Data Type Conversion/1
  Data Type Conversion1/1 -> R_HALOUTCDD_CSOP_SetSysPwrStat/1
  [VOUTP_SysPowerMode_enum] -> Data Type Conversion1/1
  Data Type Conversion2/1 -> R_HALOUTCDD_CSOP_AppNmStateReq/1(WakeReq)
  [VOUTP_NetworkReq_flg] -> Data Type Conversion2/1
  Data Type Conversion3/1 -> R_HALOUTCDD_CSOP_AppNmStateReq/2(SleepReq)
  NOT/1 -> Data Type Conversion3/1
  [VOUTP_NetworkReq_flg] -> NOT/1
  detect_change/1 -> R_HALOUTCDD_CSOP_AppNmStateReq/Enable
  [VOUTP_NetworkReq_flg] -> detect_change/1
  [VOUTP_NvWriteReqRisingEdge_flg] -> R_NVMWriteCDD_Inner_NVM_WriteOperation/Enable
  Data Type Conversion4/1 -> R_HALOUTCDD_CSOP_SleepRequest/2(WakeUpTime)
  [VOUTP_FdcSlpTime_sec] -> Data Type Conversion4/1
  [VOUTP_FdcSlpReqRisingEdge_flg] -> R_HALOUTCDD_CSOP_SleepRequest/Enable
  Unit Delay/1 -> R_WDGCDD_CSOP_Call_WDG_AppEnd/Enable
  [VOUTP_FdcSlpReqRisingEdge_flg] -> Unit Delay/1
  Unit Delay1/1 -> R_FDCCDD_Inner_CSOP_FDC_AppCallSleep/Enable
  Unit Delay2/1 -> Unit Delay1/1
  [VOUTP_FdcSlpReqRisingEdge_flg] -> Unit Delay2/1
  [Header_Array] -> R_UDSCDD_CSOP_SetDTCStatus/1(Header_Array)
  [DTC_Array] -> R_UDSCDD_CSOP_SetDTCStatus/2(DTC_Array)
  [DTC_Trigger] -> R_UDSCDD_CSOP_SetDTCStatus/Enable
  [trig_Read_NVM_00] -> R_NVMReadCDD_Inner_NVM_ReadOperation/Trigger
  [trig_WDG] -> R_WDGCDD_CSOP_Call_Watchdog/Trigger
  detect_Increase/1 -> R_WDGCDD_CSOP_Call_WDG_AppStart/Enable
  Constant4/1 -> detect_Increase/1
  [trig_ReadIMUOffset_00] -> R_HALIN_IMU_CSOP_IMUGetOffsetVal/Trigger
  R_HALIN_IMU_CSOP_IMUGetOffsetVal/1(Out1) -> [s16_IMUOffsetVal]
  R_HALIN_IMU_CSOP_IMUGetOffsetVal/2(Out2) -> [u8_IMUOffsetValSta]
  [E2E_CAN3_VCU1_Trigger] -> HALOUT_AFTER/1(E2E_CAN3_VCU1_Trigger)
  [E2E_CAN4_VCU1_Trigger] -> HALOUT_AFTER/2(E2E_CAN4_VCU1_Trigger)
  [trig_HAL_OUTAFTER_50_1] -> HALOUT_AFTER/Trigger
  [BOUTP_DIDSetData_outputs] -> DID_CDDSubsystem/1(BOUTP_DIDSetData_outputs)
  [trig_GetDID] -> DID_CDDSubsystem/Trigger
  DID_CDDSubsystem/1(BHAL_DIDGetData_raw) -> [BHAL_DIDGetData_raw]
  hcu_main_sched/3(trig_WDG()) -> [trig_WDG]
  INP/8 -> APP/8
  [trig_HAL_IN_10] -> HAL_IN/Trigger
  HAL_IN/1 -> INP/1
  APP/10 -> OUTP/10
  APP/15 -> OUTP/15
  APP/12 -> OUTP/12
  INP/6 -> APP/6
  OUTP/1 -> [BOUTP_outputs], HAL_OUT/1
  INP/7 -> APP/7
  hcu_main_sched/9(trig_HAL_DKC_10_3()) -> [trig_HAL_DKC_10_3]
  [trig_APP_30] -> APP/Trigger
  INP/12 -> APP/12
  INP/5 -> APP/5
  APP/2 -> OUTP/2
  INP/1 -> APP/1
  [BHAL_APM_outputs] -> INP/9
  INP/2 -> APP/2
  hcu_main_sched/6(trig_HAL_IN_10()) -> [trig_HAL_IN_10]
  [BHAL_SYS_outputs] -> INP/8
  APP/4 -> OUTP/4
  APP/3 -> OUTP/3
  [BHAL_DDM_outputs] -> INP/11
  APP/7 -> OUTP/7
  [BHAL_TPMS_outputs] -> INP/7
  INP/4 -> APP/4
  APP/11 -> OUTP/11
  APP/5 -> OUTP/5
  HAL_IN/4 -> [BHAL_CAN4_outputs], INP/4
  APP/6 -> OUTP/6
  [BHAL_DKC_outputs] -> INP/10
  HAL_IN/3 -> INP/3
  APP/13 -> OUTP/13
  APP/16 -> HAL_OUT/2
  INP/9 -> APP/9
  APP/9 -> OUTP/9
  APP/1 -> OUTP/1
  [trig_INP_20] -> INP/Trigger
  [BHAL_IMU_outputs] -> INP/12
  hcu_main_sched/13(trig_OUTP_AFTER_40_1()) -> [trig_OUTP_AFTER_40_1]
  APP/14 -> OUTP/14
  [trig_HAL_OUT_50] -> HAL_OUT/Trigger
  [s8_AcoreReadyToSleep] -> HAL_OUT/3
  HAL_IN/2 -> INP/2, [BHAL_CAN2_outputs]
  APP/8 -> OUTP/8
  hcu_main_sched/12(trig_OUTP_40()) -> [trig_OUTP_40]
  hcu_main_sched/2(trig_ReadIMUOffset_00()) -> [trig_ReadIMUOffset_00]
  [trig_OUTP_40] -> OUTP/Trigger
  INP/3 -> APP/3
  hcu_main_sched/1(trig_Read_NVM_00()) -> [trig_Read_NVM_00]
  hcu_main_sched/15(trig_HAL_OUTAFTER_50_1()) -> [trig_HAL_OUTAFTER_50_1]
  HAL_IN/5 -> INP/5
  hcu_main_sched/4(trig_GetNMID()) -> [trig_GetNMID]
  hcu_main_sched/14(trig_HAL_OUT_50()) -> [trig_HAL_OUT_50]
  hcu_main_sched/8(trig_HAL_DKC_10_2()) -> [trig_HAL_DKC_10_2]
  INP/11 -> APP/11
  hcu_main_sched/11(trig_APP_30()) -> [trig_APP_30]
  hcu_main_sched/5(trig_GetDID()) -> [trig_GetDID]
  INP/10 -> APP/10
  hcu_main_sched/7(trig_HAL_CDD_10_1()) -> [trig_HAL_CDD_10_1]
  [BHAL_GPIO_outputs] -> INP/6
  hcu_main_sched/10(trig_INP_20()) -> [trig_INP_20]
  Constant5/1 -> hcu_main_sched/1(VHAL_FusionSchedReq_flg)
  R_CAN1_ABM1_CAN1_SG_ABM1_read/1 -> HAL_IN/1
  R_CAN1_EPAS1_CAN1_SG_EPAS1_read/1 -> HAL_IN/2
  R_CAN1_EPAS2_CAN1_SG_EPAS2_read/1 -> HAL_IN/3
  R_CAN1_EPB1_CAN1_SG_EPB1_read/1 -> HAL_IN/4
  R_CAN1_ESC1_CAN1_SG_ESC1_read/1 -> HAL_IN/5
  R_CAN1_ESC2_CAN1_SG_ESC2_read/1 -> HAL_IN/6
  R_CAN1_ESC3_CAN1_SG_ESC3_read/1 -> HAL_IN/7
  R_CAN1_ESC4_CAN1_SG_ESC4_read/1 -> HAL_IN/8
  R_CAN1_ESC5_CAN1_SG_ESC5_read/1 -> HAL_IN/9
  R_CAN1_ESC6_CAN1_SG_ESC6_read/1 -> HAL_IN/10
  R_CAN1_ESC7_CAN1_SG_ESC7_read/1 -> HAL_IN/11
  R_CAN1_FCM2_CAN1_SG_FCM2_read/1 -> HAL_IN/12
  R_CAN1_FCM3_CAN1_SG_FCM3_read/1 -> HAL_IN/13
  R_CAN1_FCM4_CAN1_SG_FCM4_read/1 -> HAL_IN/14
  R_CAN1_SRR1_CAN1_SG_SRR1_read/1 -> HAL_IN/15
  R_CAN2_IVI1_CAN2_SG_IVI1_read/1 -> HAL_IN/16
  R_CAN2_IVI2_CAN2_SG_IVI2_read/1 -> HAL_IN/17
  R_CAN2_IVI6_CAN2_SG_IVI6_read/1 -> HAL_IN/18
  R_CAN2_METER1_CAN2_SG_METER1_read/1 -> HAL_IN/19
  R_CAN3_BMS1_CAN3_SG_BMS1_read/1 -> HAL_IN/20
  R_CAN3_BMS2_CAN3_SG_BMS2_read/1 -> HAL_IN/21
  R_CAN3_BMS3_CAN3_SG_BMS3_read/1 -> HAL_IN/22
  R_CAN3_BMS4_CAN3_SG_BMS4_read/1 -> HAL_IN/23
  R_CAN3_BMS6_CAN3_SG_BMS6_read/1 -> HAL_IN/24
  R_CAN3_BMS7_CAN3_SG_BMS7_read/1 -> HAL_IN/25
  R_CAN3_CCU1_CAN3_SG_CCU1_read/1 -> HAL_IN/26
  R_CAN3_CCU2_CAN3_SG_CCU2_read/1 -> HAL_IN/27
  R_CAN3_CCU4_CAN3_SG_CCU4_read/1 -> HAL_IN/28
  R_CAN3_MCU_F1_CAN3_SG_MCU_F1_read/1 -> HAL_IN/29
  R_CAN3_MCU_F2_CAN3_SG_MCU_F2_read/1 -> HAL_IN/30
  R_CAN3_MCU_R1_CAN3_SG_MCU_R1_read/1 -> HAL_IN/31
  R_CAN3_MCU_R2_CAN3_SG_MCU_R2_read/1 -> HAL_IN/32
  R_CAN3_Shifter1_CAN3_SG_Shifter1_read/1 -> HAL_IN/33
  R_CAN4_DKC1_CAN4_SG_DKC1_read/1 -> HAL_IN/34
  R_CAN4_DKC2_CAN4_SG_DKC2_read/1 -> HAL_IN/35
  R_CAN4_GW_ZDR_PTG1_CAN4_SG_GW_ZDR_PTG1_read/1 -> HAL_IN/36
  R_CAN4_GW_ZoneDR1_CAN4_SG_GW_ZoneDR1_read/1 -> HAL_IN/37
  R_CAN4_GW_ZoneDR2_CAN4_SG_GW_ZoneDR2_read/1 -> HAL_IN/38
  R_CAN4_GW_ZoneDR3_CAN4_SG_GW_ZoneDR3_read/1 -> HAL_IN/39
  R_CAN4_GW_ZoneDR4_CAN4_SG_GW_ZoneDR4_read/1 -> HAL_IN/40
  R_CAN4_GW_ZoneDR6_CAN4_SG_GW_ZoneDR6_read/1 -> HAL_IN/41
  R_CAN4_GW_ZoneFR1_CAN4_SG_GW_ZoneFR1_read/1 -> HAL_IN/42
  R_CAN4_GW_ZoneFR2_CAN4_SG_GW_ZoneFR2_read/1 -> HAL_IN/43
  R_CAN4_Zone_Dr_SCP_CAN4_SG_Zone_Dr_SCP_read/1 -> HAL_IN/44
  R_CAN4_Zone_Dr_THCM_CAN4_SG_Zone_Dr_THCM_read/1 -> HAL_IN/45
  R_CAN4_Zone_Dr_VCU_CAN4_SG_Zone_Dr_VCU_read/1 -> HAL_IN/46
  R_CAN4_Zone_Fr_THCM_CAN4_SG_Zone_Fr_THCM_read/1 -> HAL_IN/47
  R_CAN5_TBOX1_CAN5_SG_TBOX1_read/1 -> HAL_IN/48
  HAL_OUT/1 -> P_CAN1_FD_BCM1_CAN1_SG_FD_BCM1_write/1
  HAL_OUT/2 -> P_CAN1_FD_VCU1_CAN1_SG_FD_VCU1_write/1
  HAL_OUT/3 -> P_CAN1_FD_VCU4_CAN1_SG_FD_VCU4_write/1
  HAL_OUT/4 -> P_CAN2_FD_BCM1_CAN2_SG_FD_BCM1_write/1
  HAL_OUT/5 -> P_CAN2_FD_BCM2_CAN2_SG_FD_BCM2_write/1
  HAL_OUT/6 -> P_CAN2_FD_TPMS1_CAN2_SG_FD_TPMS1_write/1
  HAL_OUT/7 -> P_CAN2_FD_TPMS2_CAN2_SG_FD_TPMS2_write/1
  HAL_OUT/8 -> P_CAN2_FD_V2L1_CAN2_SG_FD_V2L1_write/1
  HAL_OUT/9 -> P_CAN2_FD_VCU0_CAN2_SG_FD_VCU0_write/1
  HAL_OUT/10 -> P_CAN2_FD_VCU1_CAN2_SG_FD_VCU1_write/1
  HAL_OUT/11 -> P_CAN2_FD_VCU4_CAN2_SG_FD_VCU4_write/1
  HAL_OUT/12 -> P_CAN2_FD_VMC1_CAN2_SG_FD_VMC1_write/1
  HAL_OUT/13 -> P_CAN3_FD_BCM1_CAN3_SG_FD_BCM1_write/1
  HAL_OUT/14 -> P_CAN3_FD_THCM2_CAN3_SG_FD_THCM2_write/1
  HAL_OUT/15 -> P_CAN3_FD_V2L1_CAN3_SG_FD_V2L1_write/1
  HAL_OUT/16 -> P_CAN4_FD_DKC1_CAN4_SG_FD_DKC1_write/1
  HAL_OUT/17 -> P_CAN4_FD_THCM2_CAN4_SG_FD_THCM2_write/1
  HAL_OUT/18 -> P_CAN5_FD_BCM1_CAN5_SG_FD_BCM1_write/1
  HAL_OUT/19 -> P_CAN5_FD_CONN1_CAN5_SG_FD_CONN1_write/1
  HAL_OUT/20 -> P_CAN5_FD_THCM2_CAN5_SG_FD_THCM2_write/1
  HAL_OUT/21 -> P_CAN5_FD_VCU0_CAN5_SG_FD_VCU0_write/1
  HAL_OUT/22 -> P_CAN5_FD_VCU1_CAN5_SG_FD_VCU1_write/1
  HAL_OUT/23 -> P_CAN5_FD_VCU4_CAN5_SG_FD_VCU4_write/1
  HAL_OUT/24 -> IRV_ms10_CAN1_SG_FD_APS3_write/1
  HAL_OUT/25 -> IRV_ms10_CAN1_SG_FD_VCU2_write/1
  HAL_OUT/26 -> IRV_ms10_CAN1_SG_FD_VCU3_write/1
  HAL_OUT/27 -> IRV_ms10_CAN2_SG_FD_APS3_write/1
  HAL_OUT/28 -> IRV_ms10_CAN2_SG_FD_VCU2_write/1
  HAL_OUT/29 -> IRV_ms10_CAN3_SG_FD_VCU0_write/1
  HAL_OUT/30 -> IRV_ms10_CAN3_SG_FD_VCU2_write/1
  HAL_OUT/31 -> IRV_ms10_CAN5_SG_FD_VCU3_write/1
  HAL_OUT/32 -> IRV_ms100_CAN1_SG_FD_THCM1_write/1
  HAL_OUT/33 -> IRV_ms100_CAN2_SG_FD_THCM1_write/1
  HAL_OUT/34 -> IRV_ms100_CAN3_SG_FD_THCM1_write/1
  HAL_OUT/35 -> IRV_ms100_CAN4_SG_FD_THCM1_write/1
  HAL_OUT/36 -> IRV_ms20_CAN1_SG_FD_APS1_write/1
  HAL_OUT/37 -> IRV_ms20_CAN1_SG_FD_APS2_write/1
  HAL_OUT/38 -> IRV_ms20_CAN2_SG_FD_APS1_write/1
  HAL_OUT/39 -> IRV_ms20_CAN2_SG_FD_APS2_write/1
  HAL_OUT/40 -> IRV_ms500_CAN2_SG_FD_VCU5_write/1
  HAL_OUT/41 -> IRV_ms500_CAN5_SG_FD_VCU5_write/1
  HAL_OUT/42 -> IRV_ms5000_CAN2_SG_FD_VCU6_write/1
  HAL_OUT/43 -> IRV_E2E_CAN3_SG_FD_VCU1_write/1
  HAL_OUT/44 -> IRV_E2E_CAN4_SG_FD_VCU1_write/1
  HAL_OUT/45 -> [VOUTP_NetworkReq_flg]
  HAL_OUT/46 -> [VOUTP_SysPowerMode_enum]
  HAL_OUT/47 -> [VOUTP_NvWriteReqRisingEdge_flg]
  HAL_OUT/48 -> [VOUTP_FdcSlpReqRisingEdge_flg]
  HAL_OUT/49 -> [VOUTP_FdcSlpTime_sec]
  HAL_OUT/50 -> [VOUTP_IVIRST_flg]
  HAL_OUT/51 -> [E2E_CAN3_VCU1_Trigger]
  HAL_OUT/52 -> [E2E_CAN4_VCU1_Trigger]
  Halin_CDD/7(BHAL_IMU_outputs) -> [BHAL_IMU_outputs]
  Halin_CDD/9(AESKey) -> Subsystem/1(In1)
  [u16_Pedal2Vol] -> Halin_CDD/10(VHAL_AccelPedal2Vol_Raw)
  [Enable_decrypt] -> Subsystem2/1(Enable_Decrypt)
  [trig_HAL_DKC_10_2] -> Subsystem/Trigger
  [u8_PwrReqOTA] -> Halin_CDD/29(VHAL_PwrReq_OTA_enum)
  OUTP_AFTER/8(DTC_Trigger) -> [DTC_Trigger]
  Subsystem2/1(BHAL_DKC_outputs) -> [BHAL_DKC_outputs]
  [u8_ClearDTCcmd] -> Halin_CDD/42(VHAL_ClearDTCcmd_flg)
  [u8Array16_ResultData] -> Subsystem2/2(u8Array16_ResultData)
  OUTP_AFTER/2(ApsOut_SendChrgPlugStaSig) -> [u8_ApsOutSendChrgPlugSta]
  [u8_ApsInSysMode] -> Halin_CDD/8(ModOperationIn)
  [u8_BrakeLamp] -> Halin_CDD/20(VHAL_BrakeLampSW_flg)
  [u8_CurrentNMState] -> Halin_CDD/28(VHAL_CurrentNmState_enum)
  [u8_GetCAAS_Sta] -> Halin_CDD/76(u8_GetCAAS_Sta)
  [u8_GetAPS_ExitCondition] -> Halin_CDD/65(u8_GetAPS_ExitCondition)
  [u8_EvccAplusPwrUpReq] -> Halin_CDD/31(VHAL_EvccAplusPwrUpReq_flg)
  OUTP_AFTER/7(HAL_NvmWriteData_raw) -> [u8Array256_NvmWriteArray]
  OUTP_AFTER/1(ApsOut_GearPosnSig) -> [u8_ApsOutGearPosnSig]
  [u8_GetAPS_Progress_PCT] -> Halin_CDD/61(u8_GetAPS_Progress_PCT)
  [u8_CAN1BusOff] -> Halin_CDD/56(VHAL_CAN1BusOff_raw)
  [u8_CTDSW] -> Halin_CDD/18(VHAL_CentralDoorLockSW_flg)
  Halin_CDD/5(BHAL_SYSTPMS_outputs) -> [BHAL_SYSTPMS_outputs]
  [u8_BootReason] -> Halin_CDD/52(VHAL_PmicBootReason_enum)
  [u8_ApsInSensorLayout] -> Halin_CDD/6(SNSRLayoutIn)
  OUTP_AFTER/3(ApsOut_SetFrSensorOnCmd) -> [u8_ApsOutSetFrSensorOnCmd]
  [BHAL_SYSTPMS_outputs] -> OUTP_AFTER/2(BHAL_SYSTPMS_outputs)
  [u8_HoodSW] -> Halin_CDD/12(VHAL_HoodSW_flg)
  OUTP_AFTER/5(ApsOut_SetVehSpdTOCmd) -> [u8_ApsOutSetVehSpdTOCmd]
  [u8_CAN2BusOff] -> Halin_CDD/57(VHAL_CAN2BusOff_raw)
  [BOUTP_outputs] -> OUTP_AFTER/1(BOUTP_outputs)
  [u16_Pedal1Vol] -> Halin_CDD/9(VHAL_AccelPedal1Vol_Raw)
  OUTP_AFTER/9(Header_Array) -> [Header_Array]
  [u8_GetAPS_HW_Ver] -> Halin_CDD/64(u8_GetAPS_HW_Ver)
  Halin_CDD/10(DKCRawData) -> Subsystem/2(In2)
  [trig_OUTP_AFTER_40_1] -> OUTP_AFTER/Trigger
  Halin_CDD/1(BHAL_APM_outputs) -> [BHAL_APM_outputs]
  [u32_WISR] -> Halin_CDD/53(VHAL_WisrBootReason_raw32)
  [BHAL_CAN4_outputs] -> Subsystem2/3(BHAL_CAN4_outputs)
  Halin_CDD/4(BHAL_TPMS_outputs) -> [BHAL_TPMS_outputs]
  [u8_ApsInSysFailSta] -> Halin_CDD/7(StaFSyaIn)
  [u8_DidStaXWD] -> Halin_CDD/33(VHAL_DidXWDSta_flg)
  [u16_AuxBattVol100mV] -> Halin_CDD/48(VHAL_AuxBattVolmV_100mV)
  [u8_PsDoorSW] -> Halin_CDD/15(VHAL_PsDoorSW_flg)
  [BHAL_DIDGetData_raw] -> Halin_CDD/54(BHAL_DIDGetData_raw)
  Halin_CDD/2(BHAL_GPIO_outputs) -> [BHAL_GPIO_outputs]
  [trig_HAL_DKC_10_3] -> Subsystem2/Trigger
  [u8_GetAPS_RQ_Display] -> Halin_CDD/62(u8_GetAPS_RQ_Display)
  Halin_CDD/6(BHAL_DDM_outputs) -> [BHAL_DDM_outputs]
  [u8Array4_HWID] -> Halin_CDD/24(u8_HWID_4byte)
  [u8_GetAPS_V_Rq_EPAS_Ctrl] -> Halin_CDD/68(u8_GetAPS_V_Rq_EPAS_Ctrl)
  [u8_GetAPS_SW_Ver] -> Halin_CDD/63(u8_GetAPS_SW_Ver)
  [u8_DidStaDKC] -> Halin_CDD/36(VHAL_DIDVCUKeyReadSta_flg)
  [s8_AcoreReadyToSleep] -> Halin_CDD/32(VHAL_AcoreReadyToSlp_flg)
  [u8_GetCAAS_VMC_Req_A] -> Halin_CDD/77(u8_GetCAAS_VMC_Req_A)
  [u8_GetAPS_Sta_System] -> Halin_CDD/67(u8_GetAPS_Sta_System)
  [u8_NvmProtectSta] -> Halin_CDD/47(VHAL_NvmProtectSta_flg)
  [u8Array33_SWID] -> Halin_CDD/26(GetSWID_data)
  [u8Array8_ApsInLevel] -> Halin_CDD/3(APSLevelData)
  [u16_Pedal1Ref5V] -> Halin_CDD/49(VHAL_Pedal1Ref5V_raw)
  [u8_TrunkHanSW] -> Halin_CDD/21(VHAL_TrunkHanSW_flg)
  [u8_RLDoorSW] -> Halin_CDD/17(VHAL_RLDoorSW_flg)
  [u8_AnyNMID] -> Halin_CDD/27(VHAL_AnyNMID_flg)
  [u8_CAN4BusOff] -> Halin_CDD/59(VHAL_CAN4BusOff_raw)
  OUTP_AFTER/10(DTC_Array) -> [DTC_Array]
  [u8_GetAPS_Rq_EPAS_Ctrl] -> Halin_CDD/69(u8_GetAPS_Rq_EPAS_Ctrl)
  [BHAL_SYS_outputs] -> OUTP_AFTER/3(BHAL_SYS_outputs)
  [u8_GetAPS_ShftPosnReq] -> Halin_CDD/74(u8_GetAPS_ShftPosnReq)
  Constant6/1 -> Halin_CDD/25(GetSWID_status)
  [u8_GetAPS_Req] -> Halin_CDD/70(u8_GetAPS_Req)
  [BHAL_CAN2_outputs] -> Halin_CDD/40(BHAL_CAN2_outputs)
  [u8_CrashSignal] -> Halin_CDD/23(VHAL_CrashSignalGPIO_flg)
  [u8_TPMSDataInSta] -> Halin_CDD/38(TPMS_DataIn_flg)
  [u8_IMUOffsetValSta] -> Halin_CDD/45(VHAL_IMUOffsetValSta_flg)
  [u8_HazardSW] -> Halin_CDD/19(VHAL_HazardSW_flg)
  [u8Array256_NvmReadArray] -> Halin_CDD/35(HAL_NvmReadData_raw)
  [u8_AcoreRebootCmd] -> Halin_CDD/55(VHAL_AcoreRebootCmd_raw)
  [u8Array8_PasInDist] -> Halin_CDD/1(PASDistanceData)
  [u8Array12_ApsInUssSta] -> Halin_CDD/4(APSFaultStaData)
  OUTP_AFTER/4(ApsOut_SetFrSensorSwTOCmd) -> [u8_ApsOutSetFrSensorSwTOCmd]
  [s16_IMUSixAxisVal] -> Halin_CDD/44(VHAL_IMUSixAxisVal_raw)
  [u16Array4_ApsInDist] -> Halin_CDD/2(APSDistanceData)
  [u8_RRDoorSW] -> Halin_CDD/16(VHAL_RRDoorSW_flg)
  [f32_GetAPS_SpeedCmd] -> Halin_CDD/73(f32_GetAPS_SpeedCmd)
  [u8_DrDoorSW] -> Halin_CDD/14(VHAL_DrDoorSW_flg)
  [u8_DidDataXWD] -> Halin_CDD/34(VHAL_DidXWDData_enum)
  OUTP_AFTER/6(ApsOut_VehSpdSig) -> [f32_ApsOutVehSpdSig]
  [u8_CAN3BusOff] -> Halin_CDD/58(VHAL_CAN3BusOff_raw)
  [trig_HAL_CDD_10_1] -> Halin_CDD/Trigger
  [u8_BrakeSW] -> Halin_CDD/11(VHAL_BrakeSWGPIO_flg)
  [VHAL_NetworkReqCalled_flg] -> Halin_CDD/51(VHAL_NetworkReqCalled_flg)
  [u8_GetAPS_VMC_Req_A] -> Halin_CDD/75(u8_GetAPS_VMC_Req_A)
  [u8_CAN5BusOff] -> Halin_CDD/60(VHAL_CAN5BusOff_raw)
  [f32_GetAPS_Angle_Target] -> Halin_CDD/66(f32_GetAPS_Angle_Target)
  [u8_ApsInPASChime] -> Halin_CDD/5(ChimeIn)
  [u8_IMUSixAxisValSta] -> Halin_CDD/46(VHAL_IMUSixAxisValSta_flg)
  [u16_Pedal2Ref5V] -> Halin_CDD/50(VHAL_Pedal2Ref5V_raw)
  [u8_SeatSW] -> Halin_CDD/22(VHAL_SeatSW_flg)
  [u8_GetAPS_DecReq_A] -> Halin_CDD/72(u8_GetAPS_DecReq_A)
  OUTP_AFTER/11(BOUTP_DIDSetData_outputs) -> [BOUTP_DIDSetData_outputs]
  [u8Array9_TPMSData] -> Halin_CDD/39(TPMS_RawData)
  [u8_TailgateSW] -> Halin_CDD/13(VHAL_TailgateSW_flg)
  [s16_IMUOffsetVal] -> Halin_CDD/43(VHAL_IMUOffsetVal_raw)
  Subsystem/1(Out1) -> [u8Array16_ResultData]
  [f32_GetAPS_DecReq] -> Halin_CDD/71(f32_GetAPS_DecReq)
  Latch/1 -> Display/1  "VHAL_AnyNMIDLatch_flg"
  [BHAL_CAN4_outputs] -> Halin_CDD/41(BHAL_CAN4_outputs)
  [u8_AllowMovThdOTA] -> Halin_CDD/30(VHAL_AllowMovThd_OTA_enum)
  Halin_CDD/8(Enable_decrypt) -> [Enable_decrypt]
  Halin_CDD/3(BHAL_SYS_outputs) -> [BHAL_SYS_outputs]
  [u8_AnyNMID] -> Latch/1
  [u8Array8_DidDataDKC] -> Halin_CDD/37(VHAL_GetDIDVCUKey_enum)
  Unit Delay3/1 -> [VHAL_NetworkReqCalled_flg]
  R_HALOUTCDD_CSOP_AppNmStateReq/1(Outport) -> Unit Delay3/1
  Real_DetectChange/1 -> R_HALIN_IMU_CSOP_IMUSetSta/Enable
  [BOUTP_outputs] -> Bus Selector1/1
  Bus Selector2/1 -> Data Type Conversion5/1  "<VOUTP_IMUEnaCmd_flg>"
  Bus Selector5/1 -> Real_DetectChange/1  "<VOUTP_IMUEnaCmd_flg>"
  Bus Selector1/1 -> R_HALOUTCDD_CSOP_SetAcoreRebootCmdACK/Enable  "<VOUTP_AcoreRebootCmdACK_flg>"
  [BOUTP_outputs] -> Bus Selector/1
  Data Type Conversion5/1 -> R_HALIN_IMU_CSOP_IMUSetSta/1(u8_IMUEnaCmd)
  Bus Selector/1 -> R_UDSCDD_CSOP_DdmRestartOperationCycle/Enable  "<VOUTP_EnterNewOperCyc_flg>"
  [BOUTP_outputs] -> Bus Selector5/1
  [BOUTP_outputs] -> Bus Selector2/1
  Bus Selector4/32 -> Data Type Conversion65/1  "<VOUTP_LatAccelTimeOut_flg>"
  Data Type Conversion46/1 -> R_HALOUT_APS_CSOP_ApsSetTimeout/14
  Bus Selector4/60 -> Terminator4/1  "<VOUTP_LRPressIndi_enum>"
  Data Type Conversion29/1 -> R_HALOUT_APS_CSOP_ApsSetData/44
  Data Type Conversion103/1 -> R_HALOUT_APS_CSOP_ApsSetData/63
  Bus Selector3/52 -> Data Type Conversion34/1  "<VOUTP_HoodSW_flg>"
  Data Type Conversion72/1 -> R_HALOUT_APS_CSOP_ApsSetTimeout/40
  Data Type Conversion82/1 -> R_HALOUT_APS_CSOP_ApsSetTimeout/47
  Data Type Conversion73/1 -> R_HALOUT_APS_CSOP_ApsSetTimeout/41
  Bus Selector4/56 -> Data Type Conversion89/1  "<VOUTP_DriverSeatBeltCmdTimeOut_flg>"
  Bus Selector4/35 -> Data Type Conversion67/1  "<VOUTP_YawRateVTimeOut_flg>"
  Bus Selector4/40 -> Data Type Conversion72/1  "<VOUTP_BrkSwVTimeOut_flg>"
  [BOUTP_outputs] -> Bus Selector4/1
  Data Type Conversion20/1 -> R_HALOUT_APS_CSOP_ApsSetData/20
  Data Type Conversion14/1 -> R_HALOUT_APS_CSOP_ApsSetData/21
  Bus Selector4/16 -> Data Type Conversion48/1  "<VOUTP_LRPulseCountVTimeOut_flg>"
  Bus Selector3/68 -> Data Type Conversion98/1  "<VOUTP_RRDoorSW_flg>"
  Bus Selector4/23 -> Data Type Conversion70/1  "<VOUTP_DriIntendTimeOut_flg>"
  Data Type Conversion54/1 -> R_HALOUT_APS_CSOP_ApsSetTimeout/18
  Bus Selector3/6 -> R_HALOUT_APS_CSOP_ApsSetData/6  "<VOUTP_LRRawWhlSpeed_kph>"
  Bus Selector4/5 -> Data Type Conversion38/1  "<VOUTP_RRRawWhlSpeedTimeOut_flg>"
  Bus Selector3/7 -> R_HALOUT_APS_CSOP_ApsSetData/7  "<VOUTP_RRRawWhlSpeed_kph>"
  Bus Selector4/58 -> Terminator2/1  "<VOUTP_LFPressIndi_enum>"
  Bus Selector4/38 -> Data Type Conversion74/1  "<VOUTP_MCPressureVTimeOut_flg>"
  Bus Selector3/66 -> Data Type Conversion100/1  "<VOUTP_PsDoorSW_flg>"
  Bus Selector3/31 -> Data Type Conversion21/1  "<VOUTP_SASSpeedValid_flg>"
  Data Type Conversion48/1 -> R_HALOUT_APS_CSOP_ApsSetTimeout/16
  Bus Selector4/21 -> Data Type Conversion53/1  "<VOUTP_RRPulseCountTimeOut_flg>"
  Data Type Conversion40/1 -> R_HALOUT_APS_CSOP_ApsSetTimeout/7
  Bus Selector3/59 -> R_HALOUT_APS_CSOP_ApsSetData/59  "<VOUTP_CAASSw_enum>"
  Bus Selector3/8 -> Data Type Conversion6/1  "<VOUTP_LFRawWhlSpeedV_flg>"
  Bus Selector3/36 -> R_HALOUT_APS_CSOP_ApsSetData/36  "<VOUTP_LatAccel_Gps>"
  Bus Selector3/72 -> R_HALOUT_APS_CSOP_ApsSetData/72  "<VOUTP_LRPressIndi_enum>"
  Bus Selector3/43 -> Data Type Conversion28/1  "<VOUTP_BrkSwSta_flg>"
  Data Type Conversion61/1 -> R_HALOUT_APS_CSOP_ApsSetTimeout/29
  Bus Selector4/37 -> Data Type Conversion69/1  "<VOUTP_LongAccelVTimeOut_flg>"
  Bus Selector3/11 -> Data Type Conversion9/1  "<VOUTP_RRRawWhlSpeedV_flg>"
  Data Type Conversion50/1 -> R_HALOUT_APS_CSOP_ApsSetTimeout/3
  Bus Selector4/12 -> Data Type Conversion45/1  "<VOUTP_LRWhlRotDirTimeOut_flg>"
  Data Type Conversion67/1 -> R_HALOUT_APS_CSOP_ApsSetTimeout/35
  Data Type Conversion93/1 -> R_HALOUT_APS_CSOP_ApsSetTimeout/59
  Bus Selector4/8 -> Data Type Conversion44/1  "<VOUTP_LRRawWhlSpeedVTimeOut_flg>"
  Bus Selector3/45 -> Data Type Conversion30/1  "<VOUTP_ESCStandstill_flg>"
  Data Type Conversion15/1 -> R_HALOUT_APS_CSOP_ApsSetData/22
  Data Type Conversion89/1 -> R_HALOUT_APS_CSOP_ApsSetTimeout/56
  Data Type Conversion65/1 -> R_HALOUT_APS_CSOP_ApsSetTimeout/32
  Data Type Conversion19/1 -> R_HALOUT_APS_CSOP_ApsSetTimeout/4
  Data Type Conversion96/1 -> R_HALOUT_APS_CSOP_ApsSetData/75
  Data Type Conversion6/1 -> R_HALOUT_APS_CSOP_ApsSetData/8
  Data Type Conversion84/1 -> R_HALOUT_APS_CSOP_ApsSetTimeout/55
  Bus Selector4/11 -> Data Type Conversion43/1  "<VOUTP_RFWhlRotDirTimeOut_flg>"
  Data Type Conversion70/1 -> R_HALOUT_APS_CSOP_ApsSetTimeout/23
  Bus Selector4/50 -> Data Type Conversion95/1  "<VOUTP_AVMErrSTATimeOut_flg>"
  Data Type Conversion69/1 -> R_HALOUT_APS_CSOP_ApsSetTimeout/37
  Data Type Conversion45/1 -> R_HALOUT_APS_CSOP_ApsSetTimeout/12
  Ground4/1 -> Data Type Conversion94/1
  Data Type Conversion87/1 -> R_HALOUT_APS_CSOP_ApsSetTimeout/52
  Data Type Conversion10/1 -> R_HALOUT_APS_CSOP_ApsSetData/16
  Data Type Conversion71/1 -> R_HALOUT_APS_CSOP_ApsSetTimeout/39
  Data Type Conversion11/1 -> R_HALOUT_APS_CSOP_ApsSetData/17
  Bus Selector3/37 -> R_HALOUT_APS_CSOP_ApsSetData/37  "<VOUTP_LongAccel_Gps>"
  Bus Selector3/29 -> R_HALOUT_APS_CSOP_ApsSetData/29  "<VOUTP_SASAngle_Deg>"
  Data Type Conversion63/1 -> R_HALOUT_APS_CSOP_ApsSetTimeout/31
  Bus Selector4/9 -> Data Type Conversion41/1  "<VOUTP_RRRawWhlSpeedVTimeOut_flg>"
  Bus Selector4/4 -> Data Type Conversion19/1  "<VOUTP_LRRawWhlSpeedTimeOut_flg>"
  Data Type Conversion38/1 -> R_HALOUT_APS_CSOP_ApsSetTimeout/5
  Ground5/1 -> Data Type Conversion106/1
  Data Type Conversion66/1 -> R_HALOUT_APS_CSOP_ApsSetTimeout/34
  Data Type Conversion59/1 -> R_HALOUT_APS_CSOP_ApsSetTimeout/26
  Bus Selector4/27 -> Data Type Conversion60/1  "<VOUTP_SASSpeedValidTimeOut_flg>"
  Data Type Conversion58/1 -> R_HALOUT_APS_CSOP_ApsSetTimeout/25
  Bus Selector3/57 -> Data Type Conversion36/1  "<VOUTP_AVMErrSTA_flg>"
  Bus Selector4/46 -> Data Type Conversion79/1  "<VOUTP_EPBStaTimeOut_flg>"
  Bus Selector4/26 -> Data Type Conversion59/1  "<VOUTP_SASSpeedTimeOut_flg>"
  Bus Selector4/22 -> Data Type Conversion56/1  "<VOUTP_ShifterHandleCmdTimeOut_flg>"
  Bus Selector4/7 -> Data Type Conversion40/1  "<VOUTP_RFRawWhlSpeedVTimeOut_flg>"
  Bus Selector4/6 -> Data Type Conversion39/1  "<VOUTP_LFRawWhlSpeedVTimeOut_flg>"
  Bus Selector4/31 -> Data Type Conversion63/1  "<VOUTP_YawRateTimeOut_flg>"
  Bus Selector3/4 -> R_HALOUT_APS_CSOP_ApsSetData/4  "<VOUTP_LFRawWhlSpeed_kph>"
  Bus Selector4/24 -> Data Type Conversion57/1  "<VOUTP_EPSAOIControlTimeOut_flg>"
  Bus Selector3/47 -> Data Type Conversion31/1  "<VOUTP_EPBExtReleaseAvail_flg>"
  Bus Selector4/54 -> Data Type Conversion81/1  "<VOUTP_ABSActiveTimeOut_flg>"
  Ground2/1 -> Data Type Conversion92/1
  Bus Selector4/13 -> Data Type Conversion55/1  "<VOUTP_RRWhlRotDirTimeOut_flg>"
  Bus Selector4/48 -> Data Type Conversion83/1  "<VOUTP_AVMparkingexcuteTimeOut_flg>"
  Bus Selector3/50 -> R_HALOUT_APS_CSOP_ApsSetData/50  "<VOUTP_EPBSta_enum>"
  Bus Selector3/24 -> Data Type Conversion17/1  "<VOUTP_APSActive_flg>"
  Data Type Conversion34/1 -> R_HALOUT_APS_CSOP_ApsSetData/52
  Bus Selector3/73 -> R_HALOUT_APS_CSOP_ApsSetData/73  "<VOUTP_sigAmbAirT_C>"
  Data Type Conversion57/1 -> R_HALOUT_APS_CSOP_ApsSetTimeout/24
  Data Type Conversion17/1 -> R_HALOUT_APS_CSOP_ApsSetData/24
  Data Type Conversion51/1 -> R_HALOUT_APS_CSOP_ApsSetTimeout/19
  Bus Selector3/38 -> R_HALOUT_APS_CSOP_ApsSetData/38  "<VOUTP_MCPressure_bar>"
  Bus Selector4/51 -> Data Type Conversion86/1  "<VOUTP_IVIStatusTimeOut_flg>"
  Data Type Conversion33/1 -> R_HALOUT_APS_CSOP_ApsSetData/51
  Bus Selector3/70 -> R_HALOUT_APS_CSOP_ApsSetData/70  "<VOUTP_LFPressIndi_enum>"
  Data Type Conversion98/1 -> R_HALOUT_APS_CSOP_ApsSetData/68
  Data Type Conversion100/1 -> R_HALOUT_APS_CSOP_ApsSetData/66
  Data Type Conversion37/1 -> R_HALOUT_APS_CSOP_ApsSetData/58
  Bus Selector4/55 -> Data Type Conversion84/1  "<VOUTP_TCSActiveTimeOut_flg>"
  Data Type Conversion105/1 -> R_HALOUT_APS_CSOP_ApsSetData/61
  Data Type Conversion26/1 -> R_HALOUT_APS_CSOP_ApsSetData/41
  Bus Selector3/13 -> R_HALOUT_APS_CSOP_ApsSetData/13  "<VOUTP_RFWhlRotDir_enum>"
  Data Type Conversion32/1 -> R_HALOUT_APS_CSOP_ApsSetData/48
  Bus Selector4/30 -> Data Type Conversion62/1  "<VOUTP_GRADETimeOut_flg>"
  Bus Selector3/34 -> R_HALOUT_APS_CSOP_ApsSetData/34  "<VOUTP_GRADE_Deg>"
  Bus Selector3/55 -> R_HALOUT_APS_CSOP_ApsSetData/55  "<VOUTP_AVMparkingexcute_enum>"
  Data Type Conversion8/1 -> R_HALOUT_APS_CSOP_ApsSetData/10
  Bus Selector3/5 -> R_HALOUT_APS_CSOP_ApsSetData/5  "<VOUTP_RFRawWhlSpeed_kph>"
  Bus Selector3/3 -> R_HALOUT_APS_CSOP_ApsSetData/3  "<VOUTP_ActAPSPosn_pct>"
  Data Type Conversion104/1 -> R_HALOUT_APS_CSOP_ApsSetData/62
  Bus Selector3/28 -> R_HALOUT_APS_CSOP_ApsSetData/28  "<VOUTP_EPSAOIControl_enum>"
  Data Type Conversion25/1 -> R_HALOUT_APS_CSOP_ApsSetData/40
  Data Type Conversion99/1 -> R_HALOUT_APS_CSOP_ApsSetData/67
  Bus Selector3/30 -> R_HALOUT_APS_CSOP_ApsSetData/30  "<VOUTP_SASSpeed_degps>"
  Bus Selector3/48 -> Data Type Conversion32/1  "<VOUTP_EPBExtApplyAvail_flg>"
  Bus Selector3/69 -> R_HALOUT_APS_CSOP_ApsSetData/69  "<VOUTP_RFPressIndi_enum>"
  Bus Selector3/1 -> R_HALOUT_APS_CSOP_ApsSetData/1  "<VOUTP_PowerSta_enum>"
  Bus Selector4/28 -> Data Type Conversion64/1  "<VOUTP_SASCALTimeOut_flg>"
  Bus Selector3/23 -> Data Type Conversion16/1  "<VOUTP_RRPulseCount_enum>"
  Bus Selector4/18 -> Data Type Conversion54/1  "<VOUTP_LFPulseCountTimeOut_flg>"
  Bus Selector3/44 -> Data Type Conversion29/1  "<VOUTP_BrkSwV_flg>"
  Bus Selector3/42 -> Data Type Conversion27/1  "<VOUTP_MCPressureV_bar>"
  Bus Selector3/51 -> Data Type Conversion33/1  "<VOUTP_AllDoorSW_flg>"
  Bus Selector3/18 -> Data Type Conversion12/1  "<VOUTP_LRPulseCountV_flg>"
  Data Type Conversion7/1 -> R_HALOUT_APS_CSOP_ApsSetData/9
  Bus Selector3/16 -> Data Type Conversion10/1  "<VOUTP_LFPulseCountV_flg>"
  Bus Selector3/61 -> Data Type Conversion105/1  "<VOUTP_CAASCtrlAvail_flg>"
  Bus Selector3/62 -> Data Type Conversion104/1  "<VOUTP_ABSActive_flg>"
  Bus Selector3/58 -> Data Type Conversion37/1  "<VOUTP_IVIStatus_flg>"
  Bus Selector3/20 -> Data Type Conversion20/1  "<VOUTP_LFPulseCount_enum>"
  Bus Selector3/64 -> Data Type Conversion102/1  "<VOUTP_DriverSeatBeltCmd_flg>"
  Bus Selector3/10 -> Data Type Conversion8/1  "<VOUTP_LRRawWhlSpeedV_flg>"
  Bus Selector3/17 -> Data Type Conversion11/1  "<VOUTP_RFPulseCountV_flg>"
  Data Type Conversion28/1 -> R_HALOUT_APS_CSOP_ApsSetData/43
  Bus Selector3/75 -> Data Type Conversion96/1  "<VOUTP_CAASActive_flg>"
  Bus Selector3/21 -> Data Type Conversion14/1  "<VOUTP_RFPulseCount_enum>"
  Bus Selector3/41 -> Data Type Conversion26/1  "<VOUTP_LongAccelV_flg>"
  Bus Selector3/63 -> Data Type Conversion103/1  "<VOUTP_TCSActive_flg>"
  Bus Selector3/9 -> Data Type Conversion7/1  "<VOUTP_RFRawWhlSpeedV_flg>"
  Bus Selector3/53 -> Data Type Conversion35/1  "<VOUTP_TailgateSW_flg>"
  Bus Selector3/2 -> R_HALOUT_APS_CSOP_ApsSetData/2  "<VOUTP_BrkPedalPos_pct>"
  Bus Selector3/49 -> R_HALOUT_APS_CSOP_ApsSetData/49  "<VOUTP_EPBErrSta_enum>"
  Bus Selector3/65 -> Data Type Conversion101/1  "<VOUTP_DrDoorSW_flg>"
  Bus Selector3/46 -> R_HALOUT_APS_CSOP_ApsSetData/46  "<VOUTP_ESCAPSSta_enum>"
  Data Type Conversion23/1 -> R_HALOUT_APS_CSOP_ApsSetData/33
  Bus Selector3/32 -> Data Type Conversion22/1  "<VOUTP_SASCAL_flg>"
  [BOUTP_outputs] -> Bus Selector3/1
  Bus Selector3/54 -> R_HALOUT_APS_CSOP_ApsSetData/54  "<VOUTP_AVMparkingcancel_enum>"
  Bus Selector4/15 -> Data Type Conversion47/1  "<VOUTP_RFPulseCountVTimeOut_flg>"
  Data Type Conversion21/1 -> R_HALOUT_APS_CSOP_ApsSetData/31
  Bus Selector3/14 -> R_HALOUT_APS_CSOP_ApsSetData/14  "<VOUTP_LRWhlRotDir_enum>"
  Bus Selector3/22 -> Data Type Conversion15/1  "<VOUTP_LRPulseCount_enum>"
  Bus Selector3/56 -> R_HALOUT_APS_CSOP_ApsSetData/56  "<VOUTP_AVMParkingmode_enum>"
  Data Type Conversion9/1 -> R_HALOUT_APS_CSOP_ApsSetData/11
  Data Type Conversion16/1 -> R_HALOUT_APS_CSOP_ApsSetData/23
  Data Type Conversion101/1 -> R_HALOUT_APS_CSOP_ApsSetData/65
  Bus Selector4/2 -> Data Type Conversion123/1  "<VOUTP_LFRawWhlSpeedTimeOut_flg>"
  Bus Selector3/60 -> R_HALOUT_APS_CSOP_ApsSetData/60  "<VOUTP_IVIScreen_enum>"
  Bus Selector3/74 -> R_HALOUT_APS_CSOP_ApsSetData/74  "<VOUTP_VehActSpd_kph>"
  Bus Selector3/12 -> R_HALOUT_APS_CSOP_ApsSetData/12  "<VOUTP_LFWhlRotDir_enum>"
  Data Type Conversion36/1 -> R_HALOUT_APS_CSOP_ApsSetData/57
  Data Type Conversion12/1 -> R_HALOUT_APS_CSOP_ApsSetData/18
  Data Type Conversion24/1 -> R_HALOUT_APS_CSOP_ApsSetData/39
  Bus Selector3/27 -> R_HALOUT_APS_CSOP_ApsSetData/27  "<VOUTP_DriIntend_enum>"
  Bus Selector3/26 -> R_HALOUT_APS_CSOP_ApsSetData/26  "<VOUTP_ShifterHandleCmd_enum>"
  Bus Selector4/42 -> Data Type Conversion76/1  "<VOUTP_ESCAPSStaTimeOut_flg>"
  Bus Selector4/19 -> Data Type Conversion51/1  "<VOUTP_RFPulseCountTimeOut_flg>"
  Ground1/1 -> Data Type Conversion91/1
  Bus Selector4/20 -> Data Type Conversion52/1  "<VOUTP_LRPulseCountTimeOut_flg>"
  Bus Selector3/40 -> Data Type Conversion25/1  "<VOUTP_LatAccelV_flg>"
  Bus Selector4/3 -> Data Type Conversion50/1  "<VOUTP_RFRawWhlSpeedTimeOut_flg>"
  Bus Selector4/10 -> Data Type Conversion42/1  "<VOUTP_LFWhlRotDirTimeOut_flg>"
  Data Type Conversion106/1 -> R_HALOUT_APS_CSOP_ApsSetTimeout/57
  Bus Selector3/33 -> Data Type Conversion23/1  "<VOUTP_SASV_flg>"
  Bus Selector3/67 -> Data Type Conversion99/1  "<VOUTP_RLDoorSW_flg>"
  Data Type Conversion13/1 -> R_HALOUT_APS_CSOP_ApsSetData/19
  Bus Selector4/45 -> Data Type Conversion78/1  "<VOUTP_EPBErrStaTimeOut_flg>"
  Bus Selector4/25 -> Data Type Conversion58/1  "<VOUTP_SASAngleTimeOut_flg>"
  Bus Selector3/19 -> Data Type Conversion13/1  "<VOUTP_RRPulseCountV_flg>"
  Data Type Conversion22/1 -> R_HALOUT_APS_CSOP_ApsSetData/32
  Data Type Conversion76/1 -> R_HALOUT_APS_CSOP_ApsSetTimeout/42
  Data Type Conversion31/1 -> R_HALOUT_APS_CSOP_ApsSetData/47
  Bus Selector4/39 -> Data Type Conversion71/1  "<VOUTP_BrkSwStaTimeOut_flg>"
  Data Type Conversion55/1 -> R_HALOUT_APS_CSOP_ApsSetTimeout/13
  Bus Selector4/1 -> Data Type Conversion80/1  "<VOUTP_BrkPedalPosTimeOut_flg>"
  Data Type Conversion18/1 -> R_HALOUT_APS_CSOP_ApsSetData/25
  Data Type Conversion88/1 -> R_HALOUT_APS_CSOP_ApsSetTimeout/53
  Bus Selector4/29 -> Data Type Conversion61/1  "<VOUTP_SASVTimeOut_flg>"
  Bus Selector4/49 -> Data Type Conversion85/1  "<VOUTP_AVMParkingmodeTimeOut_flg>"
  Bus Selector4/43 -> Data Type Conversion90/1  "<VOUTP_EPBExtReleaseAvailTimeOut_flg>"
  Data Type Conversion85/1 -> R_HALOUT_APS_CSOP_ApsSetTimeout/49
  Bus Selector4/52 -> Data Type Conversion87/1  "<VOUTP_CAASSwTimeOut_flg>"
  Data Type Conversion27/1 -> R_HALOUT_APS_CSOP_ApsSetData/42
  Bus Selector4/53 -> Data Type Conversion88/1  "<VOUTP_IVIScreenTimeOut_flg>"
  Data Type Conversion78/1 -> R_HALOUT_APS_CSOP_ApsSetTimeout/45
  Bus Selector4/33 -> Data Type Conversion75/1  "<VOUTP_LongAccelTimeOut_flg>"
  Data Type Conversion39/1 -> R_HALOUT_APS_CSOP_ApsSetTimeout/6
  Data Type Conversion86/1 -> R_HALOUT_APS_CSOP_ApsSetTimeout/51
  Data Type Conversion35/1 -> R_HALOUT_APS_CSOP_ApsSetData/53
  Data Type Conversion41/1 -> R_HALOUT_APS_CSOP_ApsSetTimeout/9
  Data Type Conversion42/1 -> R_HALOUT_APS_CSOP_ApsSetTimeout/10
  Data Type Conversion44/1 -> R_HALOUT_APS_CSOP_ApsSetTimeout/8
  Data Type Conversion47/1 -> R_HALOUT_APS_CSOP_ApsSetTimeout/15
  Bus Selector3/39 -> Data Type Conversion24/1  "<VOUTP_YawRateV_flg>"
  Data Type Conversion90/1 -> R_HALOUT_APS_CSOP_ApsSetTimeout/43
  Data Type Conversion81/1 -> R_HALOUT_APS_CSOP_ApsSetTimeout/54
  Bus Selector4/47 -> Data Type Conversion82/1  "<VOUTP_AVMparkingcancelTimeOut_flg>"
  Data Type Conversion92/1 -> R_HALOUT_APS_CSOP_ApsSetTimeout/60
  Bus Selector4/59 -> Terminator3/1  "<VOUTP_RRPressIndi_enum>"
  Data Type Conversion95/1 -> R_HALOUT_APS_CSOP_ApsSetTimeout/50
  Bus Selector3/15 -> R_HALOUT_APS_CSOP_ApsSetData/15  "<VOUTP_RRWhlRotDir_enum>"
  Data Type Conversion52/1 -> R_HALOUT_APS_CSOP_ApsSetTimeout/20
  Data Type Conversion123/1 -> R_HALOUT_APS_CSOP_ApsSetTimeout/2
  Data Type Conversion83/1 -> R_HALOUT_APS_CSOP_ApsSetTimeout/48
  Bus Selector4/17 -> Data Type Conversion49/1  "<VOUTP_RRPulseCountVTimeOut_flg>"
  Data Type Conversion43/1 -> R_HALOUT_APS_CSOP_ApsSetTimeout/11
  Bus Selector3/35 -> R_HALOUT_APS_CSOP_ApsSetData/35  "<VOUTP_YawRate_degps>"
  Data Type Conversion91/1 -> R_HALOUT_APS_CSOP_ApsSetTimeout/61
  Bus Selector4/14 -> Data Type Conversion46/1  "<VOUTP_LFPulseCountVTimeOut_flg>"
  Bus Selector3/71 -> R_HALOUT_APS_CSOP_ApsSetData/71  "<VOUTP_RRPressIndi_enum>"
  Data Type Conversion74/1 -> R_HALOUT_APS_CSOP_ApsSetTimeout/38
  Data Type Conversion56/1 -> R_HALOUT_APS_CSOP_ApsSetTimeout/22
  Data Type Conversion64/1 -> R_HALOUT_APS_CSOP_ApsSetTimeout/28
  Bus Selector4/44 -> Data Type Conversion77/1  "<VOUTP_EPBExtApplyAvailTimeOut_flg>"
  Data Type Conversion94/1 -> R_HALOUT_APS_CSOP_ApsSetTimeout/58
  Bus Selector4/41 -> Data Type Conversion73/1  "<VOUTP_ESCStandstillTimeOut_flg>"
  Data Type Conversion30/1 -> R_HALOUT_APS_CSOP_ApsSetData/45
  Data Type Conversion80/1 -> R_HALOUT_APS_CSOP_ApsSetTimeout/1
  Data Type Conversion79/1 -> R_HALOUT_APS_CSOP_ApsSetTimeout/46
  Data Type Conversion75/1 -> R_HALOUT_APS_CSOP_ApsSetTimeout/33
  Data Type Conversion102/1 -> R_HALOUT_APS_CSOP_ApsSetData/64
  Bus Selector4/34 -> Data Type Conversion66/1  "<VOUTP_MCPressureTimeOut_flg>"
  Data Type Conversion49/1 -> R_HALOUT_APS_CSOP_ApsSetTimeout/17
  Bus Selector4/57 -> Terminator1/1  "<VOUTP_RFPressIndi_enum>"
  Bus Selector3/25 -> Data Type Conversion18/1  "<VOUTP_APSCtrlAvail_flg>"
  Bus Selector4/36 -> Data Type Conversion68/1  "<VOUTP_LatAccelVTimeOut_flg>"
  Data Type Conversion60/1 -> R_HALOUT_APS_CSOP_ApsSetTimeout/27
  Bus Selector4/61 -> Terminator5/1  "<VOUTP_sigAmbAirT_C>"
  Data Type Conversion53/1 -> R_HALOUT_APS_CSOP_ApsSetTimeout/21
  Data Type Conversion77/1 -> R_HALOUT_APS_CSOP_ApsSetTimeout/44
  Data Type Conversion68/1 -> R_HALOUT_APS_CSOP_ApsSetTimeout/36
  Data Type Conversion62/1 -> R_HALOUT_APS_CSOP_ApsSetTimeout/30
  Ground3/1 -> Data Type Conversion93/1
  R_UDSCDD_CSOP_SetDTCStatus/1(Out1) -> Terminator/1
  Ground/1 -> R_HALOUTCDD_CSOP_SleepRequest/1(SleepState)
  Subsystem1/1(Out1) -> [u8_AnyNMID]
  [trig_GetNMID] -> Subsystem1/Trigger
